simulink model "HvCoorn"  (R2022b)
settings: configuration reference "Icar05FusaMdlCfg" (kept outside this file)
undefined symbols (not defined in the file): BMSActSt_ACChrg, BMSActSt_DCChrg, BMSActSt_disconnect, BMSActSt_offline, BMSActSt_online, BMSActSt_undefined, BMSMainNegRlySt_Clsd_SC, BMSMainNegRlySt_Open_SC, BMSMainNegRlySt_StuckInClsd_SC, BMSMainNegRlySt_StuckInOpen_SC, BMSMainPosRlySt_Clsd_SC, BMSMainPosRlySt_Open_SC, BMSMainPosRlySt_StuckInClsd_SC, BMSPrecRlySt_StuckInOpen_SC, BMSReqSt_ACChrg, BMSReqSt_DCChrg, BMSReqSt_emergencyOffline, BMSReqSt_offline, BMSReqSt_online, Chrg_stCycleBookMod_SC, Chrg_stSingleBookMod_SC, CmpgMod_stInactv_SC, DCDCActSt_buck, DCDCActSt_connected, DCDCActSt_disconnected, DCDCReqSt_buck, DCDCReqSt_standby, EngStrtStop_RefuModDft_SC, EPBActSt_Appld_SC, GearLvr_stDrvGearD_SC, GearLvr_stDrvGearN_SC, GearLvr_stDrvGearP_SC, GearLvr_stDrvGearR_SC, hpp_bACChargeLinkIni_C, hpp_bACChargeLinkOKIni_C, hpp_bAcChgEnaIni_C, hpp_bAcChgPauseIni_C, hpp_bAcLinkTempErrIni_C, hpp_bBattWarmReqIni_C, hpp_bHvilHwErrIni_C, hpp_bHvilStOkIni_C, hpp_bHvRelayClsActIni_C, hpp_bHvRelayOpnActIni_C, hpp_bHvRelayStuckIni_C, hpp_bParked4ChDchgIni_C, hpp_bRemLvBatMntnReqIni_C, hpp_bStartUpReqIni_C, hpp_stHvilCanIni_C, hpp_stWarmTimeCfgRespIni_C, HvCoorn_bAuthEnaSwt_C, HvCoorn_bAuthFailSpdLimOvrd_C, HvCoorn_bAuthFailSpdLimOvrdVal_C, HvCoorn_bAuthStrt_C, HvCoorn_bBMSUnexpdDcnctFailEna_C, HvCoorn_bBuck2RdyBypDCDCEna_C, HvCoorn_bDCChrgFctCfg_C, HvCoorn_bDcChrgWkupEnaChrgLink_C, HvCoorn_bDCDcnct4ACEna_C, HvCoorn_bDCNotBuck2ShtdwnEna_C, HvCoorn_bDrvrLevNotRdyEna_C ... (+295)
libraries: ITKLib x213, simulink x61
(part 3 of 12)

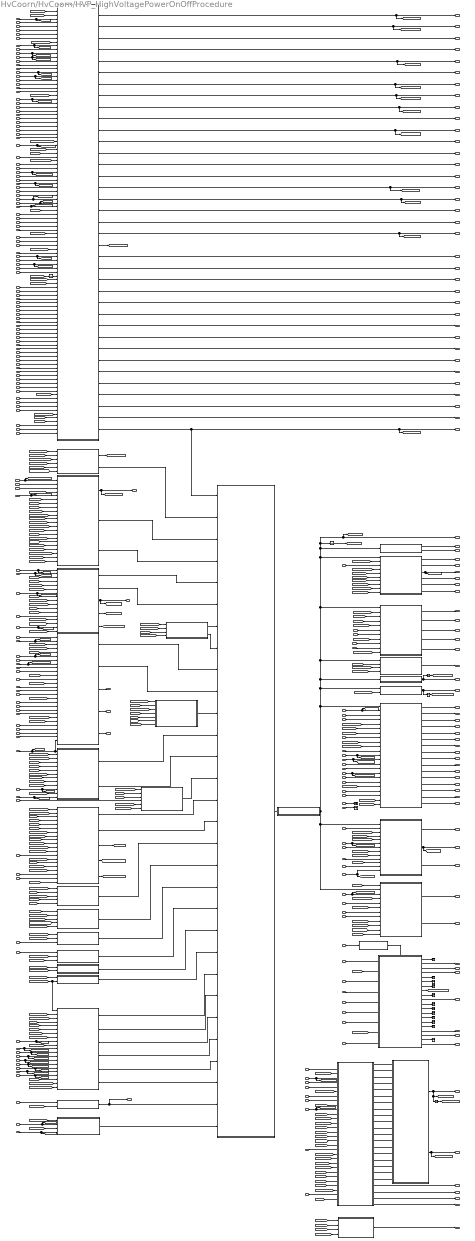
== system HvCoorn/HvCoorn/HVP_HighVoltagePowerOnOffProcedure ==
  idi_bKeyOn : Inport
  ian_uSupBattVolt : Inport  Port=2
  ian_tAcChrgrL1Temp : Inport  Port=3
  ian_tAcChrgrNTemp : Inport  Port=4
  ian_tDcChrgrTemp1 : Inport  Port=5
  ian_tDcChrgrTemp2 : Inport  Port=6
  icbms_bDcChrgWkup : Inport  Port=7
  icbms_bPrecResOverTemp : Inport  Port=8
  icbms_iHVBat : Inport  Port=9
  icbms_uHVBat : Inport  Port=10
  icbms_bBatACChrgFull : Inport  Port=11  OutDataTypeStr=boolean
  icbms_bStHvilSigErr : Inport  Port=12  OutDataTypeStr=boolean
  icbms_stHvBat : Inport  Port=13
  icbms_stHvil : Inport  Port=14  OutDataTypeStr=uint8
  icbms_stMainNegRly : Inport  Port=15  OutDataTypeStr=uint8
  icbms_stMainPosRly : Inport  Port=16  OutDataTypeStr=uint8
  icbms_stPrecRly : Inport  Port=17  OutDataTypeStr=uint8
  icbms_stDcChrgrCnct : Inport  Port=18
  icbms_bBatDCChrgFull : Inport  Port=19
  icbms_uDcChgrCap : Inport  Port=20
  icbms_iDcChgrCap : Inport  Port=21
  icecc_bStalHeatReq : Inport  Port=22
  icrm_stPlsHeatg : Inport  Port=23
  icrm_stStalHeatg : Inport  Port=24
  icbms_stDcChrg : Inport  Port=25
  icbms_bDcChrgCfg : Inport  Port=26
  icdc_bUHvActSigErr : Inport  Port=27
  icdc_stMode : Inport  Port=28
  icdc_uHvAct : Inport  Port=29
  icdc_bStHvilSigErr : Inport  Port=30  OutDataTypeStr=boolean
  icdc_stHvil : Inport  Port=31  OutDataTypeStr=uint8
  icfm_bUActSigErr : Inport  Port=32
  icfm_nAct : Inport  Port=33
  icfm_stMode : Inport  Port=34
  icfm_stActvDchrg : Inport  Port=35
  icfm_uAct : Inport  Port=36
  icrm_bUActSigErr : Inport  Port=37
  icrm_nAct : Inport  Port=38
  icrm_stMode : Inport  Port=39
  icrm_stActvDchrg : Inport  Port=40
  icrm_uAct : Inport  Port=41
  icobc_bUHvDcActSigErr : Inport  Port=42
  icobc_stChrgrCnct : Inport  Port=43
  icobc_stOBCMode : Inport  Port=44
  icobc_uHvDcAct : Inport  Port=45
  icobc_bChrgrCtrlSigCnct : Inport  Port=46  OutDataTypeStr=boolean
  icobc_bStAcHvilSigErr : Inport  Port=47  OutDataTypeStr=boolean
  icobc_pwrChrgMax : Inport  Port=48
  icobc_stHvil : Inport  Port=49  OutDataTypeStr=uint8
  icobc_uChrgrCtrlSigVolt : Inport  Port=50
  idi_bKeyStrt : Inport  Port=51
  BrkPedDev_bBrk : Inport  Port=52
  idi_bHvilInput : Inport  Port=53  OutDataTypeStr=boolean
  icacu_stWarmTime : Inport  Port=54  OutDataTypeStr=uint8
  icepb_stEpbSys : Inport  Port=55  OutDataTypeStr=uint8
  iczcu_stRmtChrgReq : Inport  Port=56
  Chrg_stBookChrgMod : Inport  Port=57  OutDataTypeStr=uint8
  ictel_stHvBatPrecdng : Inport  Port=58  OutDataTypeStr=uint8
  inv_stHvBattWarmTime : Inport  Port=59
  iud_stVCUImmo : Inport  Port=60
  iud_bNoHVHWarmTiCfg : Inport  Port=61  OutDataTypeStr=boolean
  iud_bNoHVHConfig : Inport  Port=62  OutDataTypeStr=boolean
  iud_stOBCWakeUpOrigin : Inport  Port=63  OutDataTypeStr=uint8
  iud_stRemoteImmo : Inport  Port=64  OutDataTypeStr=uint8
  PwrLimBatt_pwrMaxHvesDChrg : Inport  Port=65
  GearLvr_stDrvGear : Inport  Port=66
  VehSpd_vVeh : Inport  Port=67
  Chrg_stChrg : Inport  Port=68
  Chrg_bACChrgCmpl : Inport  Port=69  OutDataTypeStr=boolean
  Chrg_bDCChrgCmpl : Inport  Port=70
  std_tExterTemp : Inport  Port=71
  tcj_bHvBatPrecdngFinish : Inport  Port=72  OutDataTypeStr=boolean
  VehCfg_bFrntMotByp : Inport  Port=73
  Chrg_bChrgErrForever : Inport  Port=74
  icbms_bHvShutOffReq : Inport  Port=75
  iczcu_bHVPwrOffReq : Inport  Port=76
  icbms_bPlsHeatReq : Inport  Port=77
  icecc_bHVReq : Inport  Port=78
  icbms_uDCLnk : Inport  Port=79
  icbms_stPrechrgMod : Inport  Port=80
  DTC_bDiagRst : Inport  Port=81
  DTC_bDiagEnaCdnWkupLong : Inport  Port=82
  ipf_bPCAN0x130Vld : Inport  Port=83
  ipf_bPCAN0x111S1Vld : Inport  Port=84
  ipf_bPCAN0x110S1Vld : Inport  Port=85
  ipf_bPCANBusOffErr : Inport  Port=86
  icecc_bWPTCHvilFlt : Inport  Port=87
  icecc_bEASHvilFlt : Inport  Port=88
  ipf_bPCAN0x353Vld : Inport  Port=89
  DTC_bDiagEnaCdnWkupSho : Inport  Port=90
  iczcu_stFMCUAuthent : Inport  Port=91
  DrvMod_bVehShowMod : Inport  Port=92
  icicm_bPwrOffReq : Inport  Port=93
  icisg_nAct : Inport  Port=94
  ved_bInhbHvOn : Inport  Port=95
  ved_bInhbRdy : Inport  Port=96
  ved_bHvShtdwn : Inport  Port=97
  ved_bEmgcyHvShtdwn : Inport  Port=98
  ipf_bBD1CAN0x41CVld : Inport  Port=99
  icbms_stIsolTst : Inport  Port=100
  icicm_bOTAOn : Inport  Port=101
  icicm_stHVReq : Inport  Port=102
  icobc_bDchrgrCnct : Inport  Port=103
  ictcp_stRmtHvReq : Inport  Port=104
  icicm_stIvtrSwt : Inport  Port=105
  icbms_pctHVBatSOCDisp : Inport  Port=106
  icicm_pctSOCV2XLimSet : Inport  Port=107
  HvGrid_pwrMotDChrgMax : Inport  Port=108
  iczcu_stCarMod : Inport  Port=109
  ParkCtrl_bRPAActv : Inport  Port=110
  icbms_stChrgSts : Inport  Port=111
  ipf_bPCAN0x343S2Vld : Inport  Port=112
  HvCoorn_pctSOCV2XLimSetEER : Inport  Port=113
  Chrg_bChrgStopBySOCLim : Inport  Port=114
  Chrg_bBookChrgCmpl : Inport  Port=115
  iud_bNetMaintn : Inport  Port=116
  icobc_bVehCnct : Inport  Port=117
  icisg_uAct : Inport  Port=118
  icisg_stMod : Inport  Port=119
  icdkm_stLrcpReq : Inport  Port=120
  ictcp_stLostComWarn : Inport  Port=121
  iczcu_stRMCUAuthent : Inport  Port=122
  icfm_bHvilFlt : Inport  Port=123
  icrm_bHvilFlt : Inport  Port=124
  PwrLimBatt_pwrContnsDChrg : Inport  Port=125
  icicm_stIvtrEnaSwt : Inport  Port=126
  ibsw_bCnctElecDvce : Inport  Port=127
  ipf_bPCAN0x340S1Vld : Inport  Port=128
  icbms_bIsolFlt : Inport  Port=129
  DTC_bBMSFltLvlOver5 : Inport  Port=130
  icems_stEng : Inport  Port=131
  GearLvr_bNapModActv : Inport  Port=132
  GearLvr_stCmpgMod : Inport  Port=133
  GearLvr_bOffVehPwrKeep : Inport  Port=134
  GearLvr_bSentilMod : Inport  Port=135
  icebs_pctLvBatSoh : Inport  Port=136
  icbms_tMaxBat : Inport  Port=137
  icbms_tMinBat : Inport  Port=138
  icebs_tLvBat : Inport  Port=139
  icebs_pctLvBatSoc : Inport  Port=140
  icebs_stSocPrcsn : Inport  Port=141
  icebs_uLvBat : Inport  Port=142
  icicm_stOTAPwrMngtReq : Inport  Port=143
  HvCoorn_ctSmtBatMntnFailEER : Inport  Port=144
  iud_bEEIniFnsd : Inport  Port=145
  HvCoorn_ctSmtBatMntnSucsEER : Inport  Port=146
  iclbms_stLvRemChrgReq : Inport  Port=147
  ipf_bLBMSCANVld : Inport  Port=148
  VehCfg_stLvBattTyp : Inport  Port=149
  icems_nAct : Inport  Port=150
  EngStrtStop_bFuChrgActvEEW : Inport  Port=151
  icobc_stOBCModeV2In : Inport  Port=152
  icisg_bHvilFlt : Inport  Port=153
  VCU_E2_counterfaieldEER : Inport  Port=154
  VCCM_flg_Allow_Antitheft : Inport  Port=155
  VCCM_flg_Antitheft_Overtime : Inport  Port=156
  VCCM_flg_Antitheft_Start : Inport  Port=157
  ictcp_noAuthChlgOnReq : Inport  Port=158
  ictcp_noAuthSts : Inport  Port=159
  VCCM_flg_SK_Recep_ok : Inport  Port=160
  idi_uPwrSply : Inport  Port=161
  EngStrtStop_bHVPRdy : Inport  Port=162
  DTC_bBMSFltLvl6 : Inport  Port=163
  DTC_bBMSFltLvl7 : Inport  Port=164
  DTC_bBMSFltLvl8 : Inport  Port=165
  EngStrtStop_bEngStrtAllw : Inport  Port=166
  HybCoorn_bEngStrtFail : Inport  Port=167
  ved_bInhbEngStrt : Inport  Port=168
  ipf_bLIN9EBS0x34NodLostErr : Inport  Port=169
  DTC_bBMSFltLvl5 : Inport  Port=170
  EngStrtStop_stRefuMod : Inport  Port=171
  VehCfg_stCycCdn : Inport  Port=172
  icbcm_stDrvrSeatBelt : Inport  Port=173
  icbcm_bStDrvrSeatBeltSigErr : Inport  Port=174
  icbcm_bDrvrDoorAjar : Inport  Port=175
  icbcm_bDrvrDoorAjarSigErr : Inport  Port=176
  HvGrid_pwrLoadAct : Inport  Port=177
  HvCoorn_bSocWkupEER : Inport  Port=178
  HvCoorn_bTimerWkupReqEER : Inport  Port=179
  icobc_stV2LFltTyp : Inport  Port=180
  HvCoorn_stRemLvBatMntnFailRsnEER : Inport  Port=181
  icems_bFanAftRunActv : Inport  Port=182
  RngPrdn_volFuRmnByInstModEEW : Inport  Port=183
  idi_bEBSLinWkup : Inport  Port=184
  idi_bTimerWkup : Inport  Port=185
  HvCoorn_pctHVBatSocEER : Inport  Port=186
  idi_noBMSSocCounter : Inport  Port=187
  icecc_uPTCAct : Inport  Port=188
  icecc_uEASAct : Inport  Port=189
  ved_bCellVoltUndLimSrus : Inport  Port=190
  A01_HighvoltPowerUpReq : Subsystem
  A02_Init2StupCal : Subsystem  Description=初始化跳转至上高压
  A03_Comm2HVReqCal : Subsystem  Description=通讯连接跳转至高压请求
  A04_HVReq2DCBuckCal : Subsystem  Description=高压请求跳转至DCDC Buck
  A05_DCDCBuck2ReadyCal : Subsystem  Description=DCDC Buck跳转至高压Ready
  A06_ReadyWait2ReadyCal : Subsystem  Description=Ready Wait跳转至Ready
  A07_MindChange2ReadyCal : Subsystem  Description=MindChange跳转至Ready
  A08_MindChange2ShutHVCal : Subsystem  Description=MindChange跳转至断高压
  A09_ShutHV2ShutDisChCal : Subsystem  Description=断高压跳转至主动放电
  A10_ShutDisCh2ShutECUCal : Subsystem  Description=主动放电跳转至关ECU
  A11_ShutECU2AftRunCal : Subsystem  Description=关断ECU跳转至后运行
  A12_ShutECU2CommCal : Subsystem  Description=关断ECU跳转至通讯准备
  A13_AftRun2NetManCal : Subsystem  Description=后运行跳转至网络保持
  A14_NetMan2PwrShutCal : Subsystem  Description=后运行跳转至网络保持
  A15_Wake2NetManCal : Subsystem  Description=唤醒跳转至网络保持
  A16_Init2AftRunCal : Subsystem  Description=初始化跳转至后运行
  A17_EmergencyShutDownCal : Subsystem  Description=紧急下电
  A18_ShutDownReqCal : Subsystem  Description=故障下高压
  A19_MainProcedure : Stateflow chart  TreatAsAtomicUnit=on
      settings: PortSchema="{\"entries\":[{\"content\":{\"sides\":[{\"content\":{\"connectorIds\":[\"In1\",\"In2\",\"In3\",\"In4\",\"In5\",\"In6\",\"In7\",\"In8\",\"In9\",\"In10\",\"In11\",\"In12\",\"In29\",\"In13\",\"In14\",\"In15\",\"In16\",\"In17\",\"In18\",\"In19\",\"In20\",\"In21\",\"In22\",\"In23\",\"In24\",\"In25\",\"In26\",\"In27\",\"In28\",\"In30\"]},\"type\":\"ConnectorPlacement.EquallySpacedRectSide\",\"uuid\":\"b4d08740-7c56-442d-9e50-6eb0ed517615\"},{\"content\":{\"connectorIds\":[\"Out1\"],\"side\":\"RIGHT\"},\"type\":\"ConnectorPlacement.EquallySpacedRectSide\",\"uuid\":\"58ee4b8b-9875-4a72-814f-6ccb341ac7ee\"},{\"content\":{\"connectorIds\":[],\"side\":\"TOP\"},\"type\":\"ConnectorPlacement.EquallySpacedRectSide\",\"uuid\":\"584c371a-54d2-4cc4-a7a6-7136bc7e8093\"}]},\"type\":\"ConnectorPlacement.EquallySpacedConnector\",\"uuid\":\"c86f169c-7c4a-42d5-917a-7ec3533626c8\"}],\"packageUris\":[\"http://schema.mathworks.com/mf0/Connector/R2020b\"],\"version\":\"1.0\"}"
  A20_HVPStOvrd : Subsystem
  A21_ShutDwnEna : Subsystem
  A22_ModeBMSReqCal : Subsystem  Description=电池模式请求
  A23_MCUModeReqCal : Subsystem  Description=电机模式请求
  A24_DCDCModeReqCal : Subsystem  Description=DCDC模式请求
  A25_HvilClsReqCal : Subsystem
  A26_DischargeErrCal : Subsystem  Description=主动放电故障
  A27_ErrCheck : Subsystem
  A28_V2L : Subsystem
  A29_V2In : Subsystem
  A30_Authcation : Subsystem
  A30_ISGNotRdy : Subsystem
  A31_VoltModReq : Subsystem
  A32_VoltModSts : Stateflow chart  TreatAsAtomicUnit=on
  A33_ISGVoltReq : Subsystem
  Subsystem : Subsystem
  Terminator{,1..13} (14 alike) : Terminator
  Unit Delay{1..4} (4 alike) : UnitDelay  SampleTime=-1  HasFrameUpgradeWarning=on
      Unit Delay1 settings: AttributesFormatString=<initial=%<X0>>
      Unit Delay2 settings: AttributesFormatString=<initial=%<X0>>
      Unit Delay3 settings: AttributesFormatString=<initial=%<X0>>
      Unit Delay4 settings: AttributesFormatString=<initial=%<x0>>
  UnitDelay : UnitDelay  SampleTime=-1  HasFrameUpgradeWarning=on
      settings: AttributesFormatString=<Initial=%<x0>>
  HvCoorn_stHVP : Outport  VectorParamsAs1DForOutWhenUnconnected=off
  HvCoorn_stFMCUModeReq : Outport  Port=2  VectorParamsAs1DForOutWhenUnconnected=off
  HvCoorn_stRMCUModeReq : Outport  Port=3  VectorParamsAs1DForOutWhenUnconnected=off
  HvCoorn_stDCDCModeReq : Outport  Port=4  VectorParamsAs1DForOutWhenUnconnected=off
  HvCoorn_bHvOnReq : Outport  Port=5  VectorParamsAs1DForOutWhenUnconnected=off
  HvCoorn_stBMSModeReq : Outport  Port=6  VectorParamsAs1DForOutWhenUnconnected=off
  HvCoorn_bHvilClsReq : Outport  Port=7  VectorParamsAs1DForOutWhenUnconnected=off
  HvCoorn_bActvDischargeErr : Outport  Port=8  VectorParamsAs1DForOutWhenUnconnected=off
  HvCoorn_bEmgcyShutDownReq : Outport  Port=9  VectorParamsAs1DForOutWhenUnconnected=off
  HvCoorn_bHvOnFail : Outport  Port=10  VectorParamsAs1DForOutWhenUnconnected=off
  HvCoorn_bHvInitFail : Outport  Port=11  VectorParamsAs1DForOutWhenUnconnected=off
  HvCoorn_bHvReady : Outport  Port=12  VectorParamsAs1DForOutWhenUnconnected=off
  HvCoorn_bDrvRdy : Outport  Port=13  VectorParamsAs1DForOutWhenUnconnected=off
  HvCoorn_bACChrgLink : Outport  Port=14  InitialOutput=hpp_bACChargeLinkIni_C  VectorParamsAs1DForOutWhenUnconnected=off
  HvCoorn_bACChrgLinkOk : Outport  Port=15  InitialOutput=hpp_bACChargeLinkOKIni_C  VectorParamsAs1DForOutWhenUnconnected=off
  HvCoorn_stHvil : Outport  Port=16  InitialOutput=hpp_stHvilCanIni_C  VectorParamsAs1DForOutWhenUnconnected=off
  HvCoorn_bHvilHwErr : Outport  Port=17  InitialOutput=hpp_bHvilHwErrIni_C  VectorParamsAs1DForOutWhenUnconnected=off
  HvCoorn_bHvilStOk : Outport  Port=18  InitialOutput=hpp_bHvilStOkIni_C  VectorParamsAs1DForOutWhenUnconnected=off
  HvCoorn_bACChrgPause : Outport  Port=19  InitialOutput=hpp_bAcChgPauseIni_C  VectorParamsAs1DForOutWhenUnconnected=off
  HvCoorn_bStartUpReq : Outport  Port=20  InitialOutput=hpp_bStartUpReqIni_C  VectorParamsAs1DForOutWhenUnconnected=off
  HvCoorn_bHvRlyClsAct : Outport  Port=21  InitialOutput=hpp_bHvRelayClsActIni_C  VectorParamsAs1DForOutWhenUnconnected=off
  HvCoorn_bHvRlyOpenAct : Outport  Port=22  InitialOutput=hpp_bHvRelayOpnActIni_C  VectorParamsAs1DForOutWhenUnconnected=off
  HvCoorn_bHvRlyStuck : Outport  Port=23  InitialOutput=hpp_bHvRelayStuckIni_C  VectorParamsAs1DForOutWhenUnconnected=off
  HvCoorn_bACLinkTempErr : Outport  Port=24  InitialOutput=hpp_bAcLinkTempErrIni_C  VectorParamsAs1DForOutWhenUnconnected=off
  HvCoorn_bParked4ChDchg : Outport  Port=25  InitialOutput=hpp_bParked4ChDchgIni_C  VectorParamsAs1DForOutWhenUnconnected=off
  HvCoorn_bBattWarmReq : Outport  Port=26  InitialOutput=hpp_bBattWarmReqIni_C  VectorParamsAs1DForOutWhenUnconnected=off
  HvCoorn_stWarmTimeCfgResp : Outport  Port=27  InitialOutput=hpp_stWarmTimeCfgRespIni_C  VectorParamsAs1DForOutWhenUnconnected=off
  HvCoorn_bACChrgEna : Outport  Port=28  InitialOutput=hpp_bAcChgEnaIni_C  VectorParamsAs1DForOutWhenUnconnected=off
  HvCoorn_bRemLvBatMntnReq : Outport  Port=29  InitialOutput=hpp_bRemLvBatMntnReqIni_C  VectorParamsAs1DForOutWhenUnconnected=off
  HvCoorn_bDCChrgLink : Outport  Port=30  VectorParamsAs1DForOutWhenUnconnected=off
  HvCoorn_bChrgLink : Outport  Port=31  VectorParamsAs1DForOutWhenUnconnected=off
  HvCoorn_bDCLinkTempErr : Outport  Port=32  VectorParamsAs1DForOutWhenUnconnected=off
  HvCoorn_bDCChrgEna : Outport  Port=33  VectorParamsAs1DForOutWhenUnconnected=off
  HvCoorn_bRMCUPlsHeatgReq : Outport  Port=34
  HvCoorn_bRMCUStalHeatgReq : Outport  Port=35
  HvCoorn_bEccEna : Outport  Port=36  VectorParamsAs1DForOutWhenUnconnected=off
  HvCoorn_bHvRlyUnexpdDcnctErr : Outport  Port=37
  HvCoorn_bBMSUnexpdDcnctErr : Outport  Port=38
  HvCoorn_bMainRlyFail2ClsErr : Outport  Port=39
  HvCoorn_bPrechrgOvtiErr : Outport  Port=40
  HvCoorn_bDchrgOvtiErr : Outport  Port=41
  HvCoorn_bDCUnexpdDcnctErr : Outport  Port=42
  HvCoorn_stISGModeReq : Outport  Port=43  VectorParamsAs1DForOutWhenUnconnected=off
  HvCoorn_stStartUpReq : Outport  Port=44  VectorParamsAs1DForOutWhenUnconnected=off
  HvCoorn_bV2LReq : Outport  Port=45  VectorParamsAs1DForOutWhenUnconnected=off
  HvCoorn_bV2LActv : Outport  Port=46  VectorParamsAs1DForOutWhenUnconnected=off
  HvCoorn_bAllwShutNet : Outport  Port=47
  HvCoorn_bAllwSlep : Outport  Port=48
  HvCoorn_pctSOCV2XLimSetEEW : Outport  Port=49  VectorParamsAs1DForOutWhenUnconnected=off
  HvCoorn_stRdy2RdyWait : Outport  Port=50  VectorParamsAs1DForOutWhenUnconnected=off
  HvCoorn_bAuthentPass : Outport  Port=51  VectorParamsAs1DForOutWhenUnconnected=off
  HvCoorn_bBMSHvilErr : Outport  Port=52  VectorParamsAs1DForOutWhenUnconnected=off
  HvCoorn_bFMCUHvilErr : Outport  Port=53  VectorParamsAs1DForOutWhenUnconnected=off
  HvCoorn_bRMCUHvilErr : Outport  Port=54  VectorParamsAs1DForOutWhenUnconnected=off
  HvCoorn_bOBCHvilErr : Outport  Port=55  VectorParamsAs1DForOutWhenUnconnected=off
  HvCoorn_bDCDCHvilErr : Outport  Port=56  VectorParamsAs1DForOutWhenUnconnected=off
  HvCoorn_bHWHvilErr : Outport  Port=57  VectorParamsAs1DForOutWhenUnconnected=off
  HvCoorn_bWPTCHvilErr : Outport  Port=58  VectorParamsAs1DForOutWhenUnconnected=off
  HvCoorn_bEASHvilErr : Outport  Port=59  VectorParamsAs1DForOutWhenUnconnected=off
  HvCoorn_bMCUAuthentPass : Outport  Port=60  VectorParamsAs1DForOutWhenUnconnected=off
  HvCoorn_bV2InReq : Outport  Port=61  VectorParamsAs1DForOutWhenUnconnected=off
  HvCoorn_bV2InEna : Outport  Port=62  VectorParamsAs1DForOutWhenUnconnected=off
  HvCoorn_bBMSIsoErr : Outport  Port=63  VectorParamsAs1DForOutWhenUnconnected=off
  HvCoorn_bKeyOnPwrUp : Outport  Port=64  VectorParamsAs1DForOutWhenUnconnected=off
  HvCoorn_bSocWkup : Outport  Port=65  VectorParamsAs1DForOutWhenUnconnected=off
  HvCoorn_ctSmtBatMntnFailEEW : Outport  Port=66  VectorParamsAs1DForOutWhenUnconnected=off
  HvCoorn_stRemLvBatMntnFailRsn : Outport  Port=67  VectorParamsAs1DForOutWhenUnconnected=off
  HvCoorn_ctSmtBatMntnSucsEEW : Outport  Port=68  VectorParamsAs1DForOutWhenUnconnected=off
  HvCoorn_bTimerWkupReq : Outport  Port=69  VectorParamsAs1DForOutWhenUnconnected=off
  HvCoorn_bLbmsLvBatMntnReq : Outport  Port=70  VectorParamsAs1DForOutWhenUnconnected=off
  HvCoorn_pctLbmsSocMntnThd : Outport  Port=71  VectorParamsAs1DForOutWhenUnconnected=off
  HvCoorn_bLbmsSocWkup : Outport  Port=72  VectorParamsAs1DForOutWhenUnconnected=off
  HvCoorn_bISGHvilErr : Outport  Port=73  VectorParamsAs1DForOutWhenUnconnected=off
  HvCoorn_bAntiTrig430 : Outport  Port=74  VectorParamsAs1DForOutWhenUnconnected=off
  HvCoorn_bAntiTrig42C : Outport  Port=75  VectorParamsAs1DForOutWhenUnconnected=off
  VCU_E2_counterfaieldEEW : Outport  Port=76  VectorParamsAs1DForOutWhenUnconnected=off
  HvCoorn_stAuthChkFailLvl : Outport  Port=77  VectorParamsAs1DForOutWhenUnconnected=off
  HvCoorn_noVcuAuthFb : Outport  Port=78  VectorParamsAs1DForOutWhenUnconnected=off
  HvCoorn_noVcuAuthReq : Outport  Port=79  VectorParamsAs1DForOutWhenUnconnected=off
  HvCoorn_bAuthFailSpdLim : Outport  Port=80  VectorParamsAs1DForOutWhenUnconnected=off
  HvCoorn_bVehNetWkupEna : Outport  Port=81  VectorParamsAs1DForOutWhenUnconnected=off
  HvCoorn_stVoltMod : Outport  Port=82  VectorParamsAs1DForOutWhenUnconnected=off
  HvCoorn_bVoltModStbReq : Outport  Port=83  VectorParamsAs1DForOutWhenUnconnected=off
  HvCoorn_bVoltModHvDisbOvtiErr : Outport  Port=84  VectorParamsAs1DForOutWhenUnconnected=off
  HvCoorn_bVoltModHvDcnctOvtiErr : Outport  Port=85  VectorParamsAs1DForOutWhenUnconnected=off
  HvCoorn_bVoltModHvReqOvtiErr : Outport  Port=86  VectorParamsAs1DForOutWhenUnconnected=off
  HvCoorn_uISGReq : Outport  Port=87  VectorParamsAs1DForOutWhenUnconnected=off
  HvCoorn_bRdyLamp : Outport  Port=88
  HvCoorn_bSocWkupEEW : Outport  Port=89  VectorParamsAs1DForOutWhenUnconnected=off
  HvCoorn_bTimerWkupReqEEW : Outport  Port=90  VectorParamsAs1DForOutWhenUnconnected=off
  HvCoorn_stRemLvBatMntnFailRsnEEW : Outport  Port=91  VectorParamsAs1DForOutWhenUnconnected=off
  HvCoorn_pctHVBatSocEEW : Outport  Port=92  VectorParamsAs1DForOutWhenUnconnected=off
  HvCoorn_bDft2EngStrtRaw : Outport  Port=93  VectorParamsAs1DForOutWhenUnconnected=off
  HvCoorn_bShowModSocLo : Outport  Port=94  VectorParamsAs1DForOutWhenUnconnected=off
  wires:
  Unit Delay2/1 -> [HvCoorn_stHVPOld]  "HvCoorn_stHVPOld"
  [HvCoorn_stHVPOld] -> A02_Init2StupCal/5(HvCoorn_stHVPOld)
  A02_Init2StupCal/2(HvCoorn_bInit2StrtUp) -> A19_MainProcedure/2(HvCoorn_bInit2StrtUp)
  A05_DCDCBuck2ReadyCal/1(HvCoorn_bDCBuck2Rdy) -> A19_MainProcedure/7(HvCoorn_bDCBuck2Rdy)
  A07_MindChange2ReadyCal/1(HvCoorn_bMindChag2Rdy) -> A19_MainProcedure/11(HvCoorn_bMindChag2Rdy)
  A08_MindChange2ShutHVCal/1(HvCoorn_bMindChag2ShutHV) -> A19_MainProcedure/12(HvCoorn_bMindChag2ShutHV)
  A11_ShutECU2AftRunCal/1(HvCoorn_bShutECU2AftRun) -> A19_MainProcedure/16(HvCoorn_bShutECU2AftRun)
  A13_AftRun2NetManCal/1(HvCoorn_bAftRun2NetMan) -> A19_MainProcedure/18(HvCoorn_bAftRun2NetMan)
  A16_Init2AftRunCal/1(HvCoorn_bInit2AftRun) -> A19_MainProcedure/21(HvCoorn_bInit2AftRun)
  A18_ShutDownReqCal/1(HvCoorn_bEmgcyShutDownReq) -> HvCoorn_bEmgcyShutDownReq/1, A19_MainProcedure/28(HvCoorn_bEmgcyShutDownReq)
  icdc_stMode/1 -> A01_HighvoltPowerUpReq/17(icdc_stMode), [icdc_stMode]
  icfm_uAct/1 -> A04_HVReq2DCBuckCal/1(icfm_uAct), [icfm_uAct]
  [HvCoorn_bStartUpReq] -> A05_DCDCBuck2ReadyCal/2(HvCoorn_bStartUpReq)
  [HvCoorn_bStartUpReq] -> A07_MindChange2ReadyCal/1(HvCoorn_bStartUpReq)
  icbms_iHVBat/1 -> A08_MindChange2ShutHVCal/11(icbms_iHVBat), [icbms_iHVBat]
  [icfm_stMode] -> A07_MindChange2ReadyCal/2(icfm_stMode)
  [icfm_stMode] -> A08_MindChange2ShutHVCal/4(icfm_stMode)
  [icdc_stMode] -> A08_MindChange2ShutHVCal/6(icdc_stMode)
  [HvCoorn_bStartUpReq] -> A15_Wake2NetManCal/1(HvCoorn_bStartUpReq)
  [HvCoorn_bStartUpReq] -> A16_Init2AftRunCal/1(HvCoorn_bStartUpReq)
  [icfm_uAct] -> A11_ShutECU2AftRunCal/2(icfm_uAct)
  [HvCoorn_bHvRlyOpenAct] -> A17_EmergencyShutDownCal/3(HvCoorn_bHvRlyOpenAct)
  [icfm_uAct] -> A17_EmergencyShutDownCal/4(icfm_uAct)
  A25_HvilClsReqCal/1(HvCoorn_bHvilClsReq) -> Unit Delay3/1, HvCoorn_bHvilClsReq/1
  A12_ShutECU2CommCal/1(HvCoorn_bShutECU2Comm) -> A19_MainProcedure/17(HvCoorn_bShutECU2Comm)
  [HvCoorn_bStartUpReq] -> A13_AftRun2NetManCal/2(HvCoorn_bStartUpReq)
  [HvCoorn_bStartUpReq] -> A02_Init2StupCal/1(HvCoorn_bStartUpReq)
  icfm_stMode/1 -> A01_HighvoltPowerUpReq/18(icfm_stMode), [icfm_stMode]
  [icdc_uHvAct] -> A17_EmergencyShutDownCal/5(icdc_uHvAct)
  [HvCoorn_bHvRlyOpenAct] -> A09_ShutHV2ShutDisChCal/1(HvCoorn_bHvRlyOpenAct)
  idi_bKeyStrt/1 -> [idi_bKeyStrt], A06_ReadyWait2ReadyCal/2(idi_bKeyStrt)
  A23_MCUModeReqCal/1(HvCoorn_stFMCUModeReq) -> HvCoorn_stFMCUModeReq/1
  A26_DischargeErrCal/1(HvCoorn_bActvDischargeErr) -> HvCoorn_bActvDischargeErr/1, Unit Delay1/1
  A24_DCDCModeReqCal/1(HvCoorn_stDCDCModeReq) -> HvCoorn_stDCDCModeReq/1
  A22_ModeBMSReqCal/1(HvCoorn_bHvOnReq) -> HvCoorn_bHvOnReq/1
  [HvCoorn_bStartUpReq] -> A26_DischargeErrCal/2(HvCoorn_bStartUpReq)
  ian_uSupBattVolt/1 -> A03_Comm2HVReqCal/2(ian_uSupBattVolt)
  [HvCoorn_bStartUpReq] -> A08_MindChange2ShutHVCal/7(HvCoorn_bStartUpReq)
  A03_Comm2HVReqCal/2(HvCoorn_bComm2HVReq) -> A19_MainProcedure/3(HvCoorn_bComm2HVReq)
  A04_HVReq2DCBuckCal/2(HvCoorn_bHVReq2ShutDown) -> A19_MainProcedure/6(HvCoorn_bHVReq2ShutDown)
  A04_HVReq2DCBuckCal/1(HvCoorn_bHVReq2DCBuck) -> A19_MainProcedure/5(HvCoorn_bHVReq2DCBuck)
  A04_HVReq2DCBuckCal/3(HvCoorn_bHvOnFail) -> HvCoorn_bHvOnFail/1, [HvCoorn_bHvOnFail]
  A06_ReadyWait2ReadyCal/2(HvCoorn_bRdy2RdyWait) -> A19_MainProcedure/10(HvCoorn_bRdy2RdyWait)
  A06_ReadyWait2ReadyCal/1(HvCoorn_bRdyWait2Rdy) -> A19_MainProcedure/9(HvCoorn_bRdyWait2Rdy)
  A10_ShutDisCh2ShutECUCal/2(HvCoorn_bShutDisCh2ShutErr) -> A19_MainProcedure/15(HvCoorn_bShutDisCh2ShutErr)
  A10_ShutDisCh2ShutECUCal/1(HvCoorn_bShutDisCh2ShutECU) -> A19_MainProcedure/14(HvCoorn_bShutDisCh2ShutECU)
  A14_NetMan2PwrShutCal/1(HvCoorn_bNetMan2PwrShut) -> A19_MainProcedure/19(HvCoorn_bNetMan2PwrShut)
  A15_Wake2NetManCal/1(HvCoorn_bWake2NetMan) -> A19_MainProcedure/20(HvCoorn_bWake2NetMan)
  A17_EmergencyShutDownCal/5(HvCoorn_bEmWaitKeyOff2NetMan) -> A19_MainProcedure/26(HvCoorn_bEmWaitKeyOff2NetMan)
  A17_EmergencyShutDownCal/4(HvCoorn_bEmDisCh2Err) -> A19_MainProcedure/25(HvCoorn_bEmDisCh2Err)
  A17_EmergencyShutDownCal/3(HvCoorn_bEmDisCh2WaitKeyOff) -> A19_MainProcedure/24(HvCoorn_bEmDisCh2WaitKeyOff)
  A17_EmergencyShutDownCal/2(HvCoorn_bEmShutHv2DisCh) -> A19_MainProcedure/23(HvCoorn_bEmShutHv2DisCh)
  A17_EmergencyShutDownCal/1(HvCoorn_bEmIni2ShutHV) -> A19_MainProcedure/22(HvCoorn_bEmIni2ShutHV)
  icbms_bPrecResOverTemp/1 -> A03_Comm2HVReqCal/3(icbms_bPrecResOverTemp)
  GearLvr_stDrvGear/1 -> A03_Comm2HVReqCal/5(GearLvr_stDrvGear), [GearLvr_stDrvGear]
  icobc_stOBCMode/1 -> A01_HighvoltPowerUpReq/24(icobc_stOBCMode), [icobc_stOBCMode]
  [HvCoorn_bHvilStOk] -> A03_Comm2HVReqCal/11(HvCoorn_bHvilStOk)
  [HvCoorn_bStartUpReq] -> A03_Comm2HVReqCal/12(HvCoorn_bStartUpReq)
  [HvCoorn_stHVPOld] -> A03_Comm2HVReqCal/14(HvCoorn_stHVPOld)
  [HvCoorn_bObcChrgrCnct] -> A03_Comm2HVReqCal/13(HvCoorn_bObcChrgrCnct)
  icdc_uHvAct/1 -> [icdc_uHvAct], A04_HVReq2DCBuckCal/2(icdc_uHvAct)
  [HvCoorn_stHVPOld] -> A04_HVReq2DCBuckCal/6(HvCoorn_stHVPOld)
  [HvCoorn_bStartUpReq] -> A04_HVReq2DCBuckCal/9(HvCoorn_bStartUpReq)
  [icfm_stMode] -> A04_HVReq2DCBuckCal/3(icfm_stMode)
  [icdc_stMode] -> A04_HVReq2DCBuckCal/4(icdc_stMode)
  [icobc_stOBCMode] -> A04_HVReq2DCBuckCal/5(icobc_stOBCMode)
  [idi_bKeyOn] -> A04_HVReq2DCBuckCal/8(idi_bKeyOn)
  [icdc_stMode] -> A05_DCDCBuck2ReadyCal/3(icdc_stMode)
  [icobc_stOBCMode] -> A08_MindChange2ShutHVCal/8(icobc_stOBCMode)
  [HvCoorn_bStartUpReq] -> A11_ShutECU2AftRunCal/3(HvCoorn_bStartUpReq)
  [HvCoorn_bHvOnFail] -> A02_Init2StupCal/2(HvCoorn_bHvOnFail)
  Unit Delay1/1 -> [HvCoorn_bDischargeErrOld]
  [HvCoorn_bDischargeErrOld] -> A02_Init2StupCal/3(HvCoorn_bDischargeErrOld)
  idi_bKeyOn/1 -> A01_HighvoltPowerUpReq/3(idi_bKeyOn), [idi_bKeyOn]
  A22_ModeBMSReqCal/2(HvCoorn_stBMSModeReq) -> HvCoorn_stBMSModeReq/1
  A03_Comm2HVReqCal/3(HvCoorn_bComm2ShutECU) -> A19_MainProcedure/4(HvCoorn_bComm2ShutECU)
  A03_Comm2HVReqCal/1(HvCoorn_bHvInitFail) -> [HvCoorn_bHvInitFail], HvCoorn_bHvInitFail/1
  [HvCoorn_bHvInitFail] -> A02_Init2StupCal/4(HvCoorn_bHvInitFail)
  [ved_bHvShtdwn] -> A08_MindChange2ShutHVCal/9(ved_bHvShtdwn)
  icfm_nAct/1 -> A17_EmergencyShutDownCal/9(icfm_nAct), [icfm_nAct]
  [icfm_stMode] -> A17_EmergencyShutDownCal/6(icfm_stMode)
  [icfm_nAct] -> A09_ShutHV2ShutDisChCal/2(icfm_nAct)
  [HvCoorn_bStartUpReq] -> A12_ShutECU2CommCal/2(HvCoorn_bStartUpReq)
  [HvCoorn_bHvOnFail] -> A12_ShutECU2CommCal/3(HvCoorn_bHvOnFail)
  [HvCoorn_bDischargeErrOld] -> A12_ShutECU2CommCal/4(HvCoorn_bDischargeErrOld)
  A10_ShutDisCh2ShutECUCal/3(bVolDiffEnaHv) -> [bVolDiffEnaHv]
  [HvCoorn_bHvInitFail] -> A12_ShutECU2CommCal/5(HvCoorn_bHvInitFail)
  [icdc_uHvAct] -> A11_ShutECU2AftRunCal/4(icdc_uHvAct)
  [icfm_uAct] -> A10_ShutDisCh2ShutECUCal/3(icfm_uAct)
  [icdc_uHvAct] -> A10_ShutDisCh2ShutECUCal/4(icdc_uHvAct)
  [icfm_stMode] -> A10_ShutDisCh2ShutECUCal/5(icfm_stMode)
  [HvCoorn_bStartUpReq] -> A10_ShutDisCh2ShutECUCal/7(HvCoorn_bStartUpReq)
  Chrg_stChrg/1 -> A22_ModeBMSReqCal/3(Chrg_stChrg)
  [Chrg_bACChrgCmpl] -> A22_ModeBMSReqCal/5(Chrg_bACChrgCmpl)
  [HvCoorn_bACChrgLinkOk] -> A22_ModeBMSReqCal/4(HvCoorn_bACChrgLinkOk)
  [icbms_iHVBat] -> A17_EmergencyShutDownCal/7(icbms_iHVBat)
  iud_stVCUImmo/1 -> A06_ReadyWait2ReadyCal/1(iud_stVCUImmo)
  [HvCoorn_bStartUpReq] -> A06_ReadyWait2ReadyCal/4(HvCoorn_bStartUpReq)
  [idi_bKeyOn] -> A06_ReadyWait2ReadyCal/5(idi_bKeyOn)
  [HvCoorn_stHVPOld] -> A18_ShutDownReqCal/2(HvCoorn_stHVPOld)
  A01_HighvoltPowerUpReq/37(HvCoorn_bStartUpReq) -> [HvCoorn_bStartUpReq], HvCoorn_bStartUpReq/1, A19_MainProcedure/1(HvCoorn_bStartUpReq)
  [HvCoorn_bHvRlyClsAct] -> A04_HVReq2DCBuckCal/10(HvCoorn_bHvRlyClsAct)
  [HvCoorn_bHvRlyClsAct] -> A07_MindChange2ReadyCal/3(HvCoorn_bHvRlyClsAct)
  VehSpd_vVeh/1 -> A06_ReadyWait2ReadyCal/28(VehSpd_vVeh), A08_MindChange2ShutHVCal/1(VehSpd_vVeh), [VehSpd_vVeh]
  [HvCoorn_bHvRlyOpenAct] -> A08_MindChange2ShutHVCal/3(HvCoorn_bHvRlyOpenAct)
  [HvCoorn_bHvRlyOpenAct] -> A10_ShutDisCh2ShutECUCal/2(HvCoorn_bHvRlyOpenAct)
  [HvCoorn_stHVPOld] -> A08_MindChange2ShutHVCal/10(HvCoorn_stHVPOld)
  [HvCoorn_bHvRlyStuck] -> A17_EmergencyShutDownCal/2(HvCoorn_bHvRlyStuck)
  [HvCoorn_bStartUpReq] -> A17_EmergencyShutDownCal/8(HvCoorn_bStartUpReq)
  [HvCoorn_bHvRlyStuck] -> A10_ShutDisCh2ShutECUCal/14(HvCoorn_bHvRlyStuck)
  [HvCoorn_bACChrgLink] -> A22_ModeBMSReqCal/2(HvCoorn_bACChrgLink)
  [HvCoorn_bHvOnFail] -> A10_ShutDisCh2ShutECUCal/8(HvCoorn_bHvOnFail)
  A19_MainProcedure/1(HvCoorn_stHVP) -> A20_HVPStOvrd/1(HvCoorn_stHVPRaw)
  PwrLimBatt_pwrMaxHvesDChrg/1 -> A03_Comm2HVReqCal/1(PwrLimBatt_pwrMaxHvesDChrg), [PwrLimBatt_pwrMaxHvesDChrg]
  [HvCoorn_stHVPOld] -> A17_EmergencyShutDownCal/10(HvCoorn_stHVPOld)
  ved_bHvShtdwn/1 -> A17_EmergencyShutDownCal/11(ved_bHvShtdwn), [ved_bHvShtdwn]
  A17_EmergencyShutDownCal/6(HvCoorn_bEmShutHeal) -> A19_MainProcedure/27(HvCoorn_bEmShutHeal)
  icbms_uHVBat/1 -> A10_ShutDisCh2ShutECUCal/13(icbms_uHVBat)
  [bVolDiffEnaHv] -> A12_ShutECU2CommCal/1(bVolDiffEnaHv)
  icobc_uHvDcAct/1 -> [icobc_uHvDcAct], A17_EmergencyShutDownCal/12(icobc_uHvDcAct)
  icfm_bUActSigErr/1 -> [icfm_bUActSigErr], A17_EmergencyShutDownCal/13(icfm_bUActSigErr)
  icobc_bUHvDcActSigErr/1 -> [icobc_bUHvDcActSigErr], A17_EmergencyShutDownCal/14(icobc_bUHvDcActSigErr)
  icdc_bUHvActSigErr/1 -> [icdc_bUHvActSigErr], A17_EmergencyShutDownCal/15(icdc_bUHvActSigErr)
  [icobc_uHvDcAct] -> A10_ShutDisCh2ShutECUCal/9(icobc_uHvDcAct)
  [icfm_bUActSigErr] -> A10_ShutDisCh2ShutECUCal/10(icfm_bUActSigErr)
  [icobc_bUHvDcActSigErr] -> A10_ShutDisCh2ShutECUCal/11(icobc_bUHvDcActSigErr)
  [icdc_bUHvActSigErr] -> A10_ShutDisCh2ShutECUCal/12(icdc_bUHvActSigErr)
  [HvCoorn_bChrgLink] -> A06_ReadyWait2ReadyCal/3(HvCoorn_bChrgLink)
  [VehSpd_vVeh] -> A24_DCDCModeReqCal/2(VehSpd_vVeh)
  A01_HighvoltPowerUpReq/15(HvCoorn_bRemLvBatMntnReq) -> HvCoorn_bRemLvBatMntnReq/1
  Chrg_stBookChrgMod/1 -> A01_HighvoltPowerUpReq/28(Chrg_stBookChrgMod)
  A01_HighvoltPowerUpReq/6(HvCoorn_bACChrgPause) -> HvCoorn_bACChrgPause/1
  icdc_bStHvilSigErr/1 -> A01_HighvoltPowerUpReq/15(icdc_bStHvilSigErr)
  ian_tAcChrgrNTemp/1 -> A01_HighvoltPowerUpReq/5(ian_tAcChrgrNTemp)
  icacu_stWarmTime/1 -> A01_HighvoltPowerUpReq/6(icacu_stWarmTime)
  icdc_stHvil/1 -> A01_HighvoltPowerUpReq/16(icdc_stHvil)
  icobc_bStAcHvilSigErr/1 -> A01_HighvoltPowerUpReq/20(icobc_bStAcHvilSigErr)
  icbms_stHvil/1 -> A01_HighvoltPowerUpReq/11(icbms_stHvil)
  A01_HighvoltPowerUpReq/5(HvCoorn_bHvilStOk) -> [HvCoorn_bHvilStOk], HvCoorn_bHvilStOk/1
  tcj_bHvBatPrecdngFinish/1 -> A01_HighvoltPowerUpReq/41(tcj_bHvBatPrecdngFinish)
  idi_bHvilInput/1 -> A01_HighvoltPowerUpReq/30(idi_bHvilInput)
  iud_stRemoteImmo/1 -> A01_HighvoltPowerUpReq/34(iud_stRemoteImmo)
  icobc_pwrChrgMax/1 -> A01_HighvoltPowerUpReq/21(icobc_pwrChrgMax)
  A01_HighvoltPowerUpReq/2(HvCoorn_bACChrgLinkOk) -> [HvCoorn_bACChrgLinkOk], HvCoorn_bACChrgLinkOk/1
  A01_HighvoltPowerUpReq/4(HvCoorn_bHvilHwStOk) -> HvCoorn_bHvilHwErr/1
  A01_HighvoltPowerUpReq/8(HvCoorn_bHvRlyOpenAct) -> [HvCoorn_bHvRlyOpenAct], HvCoorn_bHvRlyOpenAct/1
  std_tExterTemp/1 -> A01_HighvoltPowerUpReq/39(std_tExterTemp)
  A01_HighvoltPowerUpReq/7(HvCoorn_bHvRlyClsAct) -> [HvCoorn_bHvRlyClsAct], HvCoorn_bHvRlyClsAct/1
  A01_HighvoltPowerUpReq/12(HvCoorn_bBattWarmReq) -> HvCoorn_bBattWarmReq/1
  icbms_bBatACChrgFull/1 -> A01_HighvoltPowerUpReq/7(icbms_bBatACChrgFull)
  ian_tAcChrgrL1Temp/1 -> A01_HighvoltPowerUpReq/4(ian_tAcChrgrL1Temp)
  A01_HighvoltPowerUpReq/10(HvCoorn_bACLinkTempErr) -> HvCoorn_bACLinkTempErr/1
  ictel_stHvBatPrecdng/1 -> A01_HighvoltPowerUpReq/29(ictel_stHvBatPrecdng)
  icepb_stEpbSys/1 -> A01_HighvoltPowerUpReq/26(icepb_stEpbSys)
  icbms_stMainNegRly/1 -> A01_HighvoltPowerUpReq/12(icbms_stMainNegRly), [icbms_stMainNegRly]
  icbms_stPrecRly/1 -> A01_HighvoltPowerUpReq/14(icbms_stPrecRly)
  A01_HighvoltPowerUpReq/13(HvCoorn_stWarmTimeCfgResp) -> HvCoorn_stWarmTimeCfgResp/1
  iud_bNoHVHWarmTiCfg/1 -> A01_HighvoltPowerUpReq/31(iud_bNoHVHWarmTiCfg)
  A01_HighvoltPowerUpReq/1(HvCoorn_bACChrgLink) -> [HvCoorn_bACChrgLink], HvCoorn_bACChrgLink/1
  A01_HighvoltPowerUpReq/11(HvCoorn_bParked4ChDchg) -> [HvCoorn_bParked4ChDchg], HvCoorn_bParked4ChDchg/1
  icobc_stHvil/1 -> A01_HighvoltPowerUpReq/22(icobc_stHvil)
  iud_stOBCWakeUpOrigin/1 -> A01_HighvoltPowerUpReq/33(iud_stOBCWakeUpOrigin)
  A01_HighvoltPowerUpReq/9(HvCoorn_bHvRlyStuck) -> [HvCoorn_bHvRlyStuck], HvCoorn_bHvRlyStuck/1
  icobc_uChrgrCtrlSigVolt/1 -> A01_HighvoltPowerUpReq/25(icobc_uChrgrCtrlSigVolt)
  iczcu_stRmtChrgReq/1 -> A01_HighvoltPowerUpReq/27(iczcu_stRmtChrgReq)
  icbms_bStHvilSigErr/1 -> A01_HighvoltPowerUpReq/8(icbms_bStHvilSigErr)
  iud_bNoHVHConfig/1 -> A01_HighvoltPowerUpReq/32(iud_bNoHVHConfig)
  A01_HighvoltPowerUpReq/3(HvCoorn_stHvil) -> HvCoorn_stHvil/1
  icbms_stMainPosRly/1 -> [icbms_stMainPosRly], A01_HighvoltPowerUpReq/13(icbms_stMainPosRly)
  A01_HighvoltPowerUpReq/14(HvCoorn_bACChrgEna) -> HvCoorn_bACChrgEna/1
  icobc_bChrgrCtrlSigCnct/1 -> A01_HighvoltPowerUpReq/19(icobc_bChrgrCtrlSigCnct)
  icbms_stHvBat/1 -> [icbms_stHvBat], A01_HighvoltPowerUpReq/10(icbms_stHvBat)
  [icobc_stOBCMode] -> A03_Comm2HVReqCal/9(icobc_stOBCMode)
  [icdc_stMode] -> A03_Comm2HVReqCal/7(icdc_stMode)
  [PwrLimBatt_pwrMaxHvesDChrg] -> A01_HighvoltPowerUpReq/35(PwrLimBatt_pwrMaxHvesDChrg)
  Chrg_bACChrgCmpl/1 -> A01_HighvoltPowerUpReq/36(Chrg_bACChrgCmpl), [Chrg_bACChrgCmpl]
  [idi_bKeyOn] -> A03_Comm2HVReqCal/15(idi_bKeyOn)
  [HvCoorn_bObcChrgrCnct] -> A01_HighvoltPowerUpReq/23(HvCoorn_bObcChrgrCnct)
  [GearLvr_stDrvGear] -> A01_HighvoltPowerUpReq/37(GearLvr_stDrvGear)
  [VehSpd_vVeh] -> A01_HighvoltPowerUpReq/38(VehSpd_vVeh)
  [HvCoorn_bHvilClsReqOld] -> A01_HighvoltPowerUpReq/40(HvCoorn_bHvilClsReqOld)
  [HvCoorn_tiHVPStTimer] -> A03_Comm2HVReqCal/10(HvCoorn_tiHVPStTimer)
  inv_stHvBattWarmTime/1 -> A01_HighvoltPowerUpReq/42(inv_stHvBattWarmTime)
  [icbms_pctHVBatSOCDisp] -> A03_Comm2HVReqCal/4(icbms_pctHVBatSOCDisp)
  icbms_stDcChrgrCnct/1 -> A01_HighvoltPowerUpReq/43(icbms_stDcChrgrCnct), [icbms_stDcChrgrCnct]
  ian_tDcChrgrTemp1/1 -> A01_HighvoltPowerUpReq/44(ian_tDcChrgrTemp1)
  ian_tDcChrgrTemp2/1 -> A01_HighvoltPowerUpReq/45(ian_tDcChrgrTemp2)
  Chrg_bDCChrgCmpl/1 -> A01_HighvoltPowerUpReq/46(Chrg_bDCChrgCmpl), [Chrg_bDCChrgCmpl]
  icbms_bBatDCChrgFull/1 -> A01_HighvoltPowerUpReq/47(icbms_bBatDCChrgFull)
  icbms_uDcChgrCap/1 -> A01_HighvoltPowerUpReq/48(icbms_uDcChgrCap)
  icbms_iDcChgrCap/1 -> A01_HighvoltPowerUpReq/49(icbms_iDcChgrCap)
  icbms_bDcChrgCfg/1 -> A01_HighvoltPowerUpReq/50(icbms_bDcChrgCfg), [icbms_bDcChrgCfg]
  A01_HighvoltPowerUpReq/16(HvCoorn_bDCChrgLink) -> [HvCoorn_bDCChrgLink], HvCoorn_bDCChrgLink/1
  A01_HighvoltPowerUpReq/17(HvCoorn_bChrgLink) -> [HvCoorn_bChrgLink], HvCoorn_bChrgLink/1
  A01_HighvoltPowerUpReq/18(HvCoorn_bDCLinkTempErr) -> HvCoorn_bDCLinkTempErr/1
  A01_HighvoltPowerUpReq/19(HvCoorn_bDCChrgEna) -> HvCoorn_bDCChrgEna/1
  [HvCoorn_tiHVPStTimer] -> A05_DCDCBuck2ReadyCal/1(HvCoorn_tiHVPStTimer)
  [HvCoorn_tiHVPStTimer] -> A08_MindChange2ShutHVCal/2(HvCoorn_tiHVPStTimer)
  [HvCoorn_tiHVPStTimer] -> A10_ShutDisCh2ShutECUCal/1(HvCoorn_tiHVPStTimer)
  [HvCoorn_tiHVPStTimer] -> A11_ShutECU2AftRunCal/1(HvCoorn_tiHVPStTimer)
  [HvCoorn_tiHVPStTimer] -> A13_AftRun2NetManCal/1(HvCoorn_tiHVPTimer)
  [HvCoorn_tiHVPStTimer] -> A15_Wake2NetManCal/2(HvCoorn_tiHVPTimer)
  [HvCoorn_tiHVPStTimer] -> A16_Init2AftRunCal/2(HvCoorn_tiHVPTimer), A17_EmergencyShutDownCal/1(HvCoorn_tiHVPStTimer)
  A02_Init2StupCal/1(HvCoorn_tiHVPStTimer) -> [HvCoorn_tiHVPStTimer]
  [icbms_stHvBat] -> A03_Comm2HVReqCal/6(icbms_stHvBat)
  [icfm_stMode] -> A03_Comm2HVReqCal/8(icfm_stMode)
  [HvCoorn_bDCChrgLink] -> A03_Comm2HVReqCal/16(HvCoorn_bDCChrgLink)
  A09_ShutHV2ShutDisChCal/1(HvCoorn_bShutHV2ShutDisCh) -> A19_MainProcedure/13(HvCoorn_bShutHV2ShutDisCh)
  [icbms_bDcChrgCfg] -> A22_ModeBMSReqCal/6(icbms_bDcChrgCfg)
  [Chrg_bDCChrgCmpl] -> A22_ModeBMSReqCal/7(Chrg_bDCChrgCmpl)
  A22_ModeBMSReqCal/3(HvCoorn_bHvReady) -> [HvCoorn_bHvReady], HvCoorn_bHvReady/1
  Unit Delay3/1 -> [HvCoorn_bHvilClsReqOld]
  A23_MCUModeReqCal/2(HvCoorn_stRMCUModeReq) -> HvCoorn_stRMCUModeReq/1
  icrm_nAct/1 -> [icrm_nAct], A17_EmergencyShutDownCal/16(icrm_nAct)
  icrm_uAct/1 -> [icrm_uAct], A17_EmergencyShutDownCal/18(icrm_uAct)
  [icrm_uAct] -> A04_HVReq2DCBuckCal/11(icrm_uAct)
  icrm_bUActSigErr/1 -> [icrm_bUActSigErr], A17_EmergencyShutDownCal/17(icrm_bUActSigErr)
  [icrm_bUActSigErr] -> A10_ShutDisCh2ShutECUCal/16(icrm_bUActSigErr)
  [icrm_nAct] -> A09_ShutHV2ShutDisChCal/3(icrm_nAct)
  icrm_stMode/1 -> [icrm_stMode], A01_HighvoltPowerUpReq/51(icrm_stMode)
  [icrm_stMode] -> A03_Comm2HVReqCal/17(icrm_stMode)
  [icrm_stMode] -> A04_HVReq2DCBuckCal/12(icrm_stMode)
  [icrm_stMode] -> A07_MindChange2ReadyCal/4(icrm_stMode)
  [icrm_stMode] -> A08_MindChange2ShutHVCal/5(icrm_stMode)
  [icrm_stMode] -> A10_ShutDisCh2ShutECUCal/6(icrm_stMode)
  [icrm_stMode] -> A17_EmergencyShutDownCal/19(icrm_stMode)
  [icrm_uAct] -> A10_ShutDisCh2ShutECUCal/15(icrm_uAct)
  [icrm_uAct] -> A11_ShutECU2AftRunCal/5(icrm_uAct)
  VehCfg_bFrntMotByp/1 -> A01_HighvoltPowerUpReq/52(VehCfg_bFrntMotByp), [VehCfg_bFrntMotByp]
  [VehCfg_bFrntMotByp] -> A08_MindChange2ShutHVCal/12(VehCfg_bFrntMotByp)
  [VehCfg_bFrntMotByp] -> A10_ShutDisCh2ShutECUCal/17(VehCfg_bFrntMotByp)
  [VehCfg_bFrntMotByp] -> A23_MCUModeReqCal/2(VehCfg_bFrntMotByp)
  [idi_bKeyStrt] -> A01_HighvoltPowerUpReq/53(idi_bKeyStrt)
  icfm_stActvDchrg/1 -> A10_ShutDisCh2ShutECUCal/18(icfm_stActvDchrg)
  icrm_stActvDchrg/1 -> A10_ShutDisCh2ShutECUCal/19(icrm_stActvDchrg)
  A10_ShutDisCh2ShutECUCal/4(HvCoorn_bMCUActvDchrgCmpl) -> [HvCoorn_bMCUActvDchrgCmpl]
  A10_ShutDisCh2ShutECUCal/5(HvCoorn_bMCUActvDchrgErr) -> [HvCoorn_bMCUActvDchrgErr]
  [HvCoorn_bMCUActvDchrgCmpl] -> A17_EmergencyShutDownCal/20(HvCoorn_bMCUActvDchrgCmpl)
  [HvCoorn_bMCUActvDchrgErr] -> A17_EmergencyShutDownCal/21(HvCoorn_bMCUActvDchrgErr)
  A22_ModeBMSReqCal/4(HvCoorn_bDrvRdy) -> HvCoorn_bDrvRdy/1
  [GearLvr_stDrvGear] -> A22_ModeBMSReqCal/8(GearLvr_stDrvGear)
  BrkPedDev_bBrk/1 -> [BrkPedDev_bBrk], A06_ReadyWait2ReadyCal/6(BrkPedDev_bBrk)
  icbms_bDcChrgWkup/1 -> A01_HighvoltPowerUpReq/54(icbms_bDcChrgWkup)
  [HvCoorn_bHvReady] -> A01_HighvoltPowerUpReq/1(HvCoorn_bHvReady)
  [BrkPedDev_bBrk] -> A01_HighvoltPowerUpReq/2(BrkPedDev_bBrk)
  Chrg_bChrgErrForever/1 -> A01_HighvoltPowerUpReq/55(Chrg_bChrgErrForever)
  icbms_stDcChrg/1 -> A04_HVReq2DCBuckCal/13(icbms_stDcChrg)
  [icbms_stDcChrgrCnct] -> A04_HVReq2DCBuckCal/14(icbms_stDcChrgrCnct)
  [HvCoorn_stHVPOld] -> A05_DCDCBuck2ReadyCal/4(HvCoorn_stHVPOld)
  A05_DCDCBuck2ReadyCal/2(HvCoorn_bDCBuck2Shtdwn) -> A19_MainProcedure/8(HvCoorn_bDCBuck2Shtdwn)
  [icbms_stHvBat] -> A23_MCUModeReqCal/3(icbms_stHvBat)
  [VehSpd_vVeh] -> A23_MCUModeReqCal/4(VehSpd_vVeh)
  [GearLvr_stDrvGear] -> A23_MCUModeReqCal/5(GearLvr_stDrvGear)
  icecc_bStalHeatReq/1 -> A23_MCUModeReqCal/6(icecc_bStalHeatReq)
  icrm_stPlsHeatg/1 -> A23_MCUModeReqCal/7(icrm_stPlsHeatg)
  A23_MCUModeReqCal/3(HvCoorn_bRMCUPlsHeatgReq) -> HvCoorn_bRMCUPlsHeatgReq/1
  [HvCoorn_bChrgLink] -> A23_MCUModeReqCal/8(HvCoorn_bChrgLink)
  icrm_stStalHeatg/1 -> A23_MCUModeReqCal/9(icrm_stStalHeatg)
  A23_MCUModeReqCal/4(HvCoorn_bRMCUStalHeatgReq) -> HvCoorn_bRMCUStalHeatgReq/1
  icbms_bHvShutOffReq/1 -> A01_HighvoltPowerUpReq/56(icbms_bHvShutOffReq)
  iczcu_bHVPwrOffReq/1 -> A01_HighvoltPowerUpReq/57(iczcu_bHVPwrOffReq)
  icbms_bPlsHeatReq/1 -> A23_MCUModeReqCal/10(icbms_bPlsHeatReq)
  icecc_bHVReq/1 -> A01_HighvoltPowerUpReq/58(icecc_bHVReq)
  A22_ModeBMSReqCal/5(HvCoorn_bEccEna) -> HvCoorn_bEccEna/1
  [HvCoorn_stHVPOld] -> A01_HighvoltPowerUpReq/59(HvCoorn_stHVPOld)
  A08_MindChange2ShutHVCal/2(HvCoorn_bVehSpd4HvDown) -> A19_MainProcedure/29(HvCoorn_bVehSpd4HvDown)
  [HvCoorn_bHvRlyOpenAct] -> A27_ErrCheck/5(HvCoorn_bHvRlyOpenAct)
  icbms_uDCLnk/1 -> A27_ErrCheck/4(icbms_uDCLnk)
  [icfm_uAct] -> A27_ErrCheck/7(icfm_uAct)
  [icrm_uAct] -> A27_ErrCheck/6(icrm_uAct)
  icbms_stPrechrgMod/1 -> A27_ErrCheck/3(icbms_stPrechrgMod)
  DTC_bDiagRst/1 -> [DTC_bDiagRst], A27_ErrCheck/2(DTC_bDiagRst)
  A27_ErrCheck/1(HvCoorn_bHvRlyUnexpdDcnctErr) -> HvCoorn_bHvRlyUnexpdDcnctErr/1
  A27_ErrCheck/2(HvCoorn_bBMSUnexpdDcnctErr) -> HvCoorn_bBMSUnexpdDcnctErr/1
  A27_ErrCheck/3(HvCoorn_bMainRlyFail2ClsErr) -> HvCoorn_bMainRlyFail2ClsErr/1
  A27_ErrCheck/4(HvCoorn_bPrechrgOvtiErr) -> HvCoorn_bPrechrgOvtiErr/1
  A27_ErrCheck/5(HvCoorn_bDchrgOvtiErr) -> HvCoorn_bDchrgOvtiErr/1
  DTC_bDiagEnaCdnWkupLong/1 -> A27_ErrCheck/11(DTC_bDiagEnaCdnWkupLong)
  ipf_bPCAN0x130Vld/1 -> A27_ErrCheck/12(ipf_bPCAN0x130Vld), [ipf_bPCAN0x130Vld]
  ipf_bPCAN0x111S1Vld/1 -> A27_ErrCheck/13(ipf_bPCAN0x111S1Vld), [ipf_bPCAN0x111S1Vld]
  ipf_bPCAN0x110S1Vld/1 -> A27_ErrCheck/14(ipf_bPCAN0x110S1Vld)
  ipf_bPCANBusOffErr/1 -> A27_ErrCheck/15(ipf_bPCANBusOffErr)
  [HvCoorn_bCtrlrHvilErr] -> A27_ErrCheck/10(HvCoorn_bCtrlrHvilErr)
  A27_ErrCheck/7(HvCoorn_bBMSHvilErr) -> HvCoorn_bBMSHvilErr/1
  icecc_bWPTCHvilFlt/1 -> A01_HighvoltPowerUpReq/60(icecc_bWPTCHvilFlt)
  icecc_bEASHvilFlt/1 -> A01_HighvoltPowerUpReq/61(icecc_bEASHvilFlt)
  [ipf_bPCAN0x130Vld] -> A03_Comm2HVReqCal/18(ipf_bPCAN0x130Vld)
  [ipf_bPCAN0x111S1Vld] -> A03_Comm2HVReqCal/19(ipf_bPCAN0x111S1Vld)
  DTC_bDiagEnaCdnWkupSho/1 -> A27_ErrCheck/16(DTC_bDiagEnaCdnWkupSho), [DTC_bDiagEnaCdnWkupSho]
  [DTC_bDiagEnaCdnWkupSho] -> A03_Comm2HVReqCal/20(DTC_bDiagEnaCdnWkupSho)
  ipf_bPCAN0x353Vld/1 -> A27_ErrCheck/8(ipf_bPCAN0x353Vld)
  [icdc_uHvAct] -> A27_ErrCheck/9(icdc_uHvAct)
  A27_ErrCheck/6(HvCoorn_bDCUnexpdDcnctErr) -> HvCoorn_bDCUnexpdDcnctErr/1
  iczcu_stFMCUAuthent/1 -> A06_ReadyWait2ReadyCal/7(iczcu_stFMCUAuthent)
  DrvMod_bVehShowMod/1 -> [DrvMod_bVehShowMod], A06_ReadyWait2ReadyCal/8(DrvMod_bVehShowMod)
  icicm_bPwrOffReq/1 -> A01_HighvoltPowerUpReq/62(icicm_bPwrOffReq)
  icisg_nAct/1 -> A09_ShutHV2ShutDisChCal/4(icisg_nAct)
  A23_MCUModeReqCal/5(HvCoorn_stISGModeReq) -> HvCoorn_stISGModeReq/1
  ved_bInhbHvOn/1 -> A01_HighvoltPowerUpReq/73(ved_bInhbHvOn)
  ved_bInhbRdy/1 -> A06_ReadyWait2ReadyCal/9(ved_bInhbRdy)
  ved_bEmgcyHvShtdwn/1 -> A18_ShutDownReqCal/1(ved_bEmgcyHvShtdwn)
  [ved_bHvShtdwn] -> A01_HighvoltPowerUpReq/63(ved_bHvShtdwn)
  ipf_bBD1CAN0x41CVld/1 -> A01_HighvoltPowerUpReq/64(ipf_bBD1CAN0x41CVld)
  icbms_stIsolTst/1 -> A06_ReadyWait2ReadyCal/10(icbms_stIsolTst)
  icicm_bOTAOn/1 -> [icicm_bOTAOn], A01_HighvoltPowerUpReq/65(icicm_bOTAOn)
  icicm_stHVReq/1 -> A01_HighvoltPowerUpReq/66(icicm_stHVReq)
  [icicm_bOTAOn] -> A06_ReadyWait2ReadyCal/11(icicm_bOTAOn)
  icobc_bDchrgrCnct/1 -> A01_HighvoltPowerUpReq/67(icobc_bDchrgrCnct), [icobc_bDchrgrCnct]
  A01_HighvoltPowerUpReq/20(HvCoorn_stStartUpReq) -> [HvCoorn_stStartUpReq], HvCoorn_stStartUpReq/1
  ictcp_stRmtHvReq/1 -> A01_HighvoltPowerUpReq/68(ictcp_stRmtHvReq)
  [HvCoorn_bParked4ChDchg] -> A28_V2L/5(HvCoorn_bParked4ChDchg)
  [icobc_bDchrgrCnct] -> A28_V2L/4(icobc_bDchrgrCnct)
  icbms_pctHVBatSOCDisp/1 -> A28_V2L/6(icbms_pctHVBatSOCDisp), [icbms_pctHVBatSOCDisp]
  icicm_pctSOCV2XLimSet/1 -> A28_V2L/7(icicm_pctSOCV2XLimSet)
  [icobc_stOBCMode] -> A28_V2L/8(icobc_stOBCMode)
  icicm_stIvtrSwt/1 -> A28_V2L/2(icicm_stIvtrSwt)
  [HvCoorn_bDCChrgLink] -> A28_V2L/9(HvCoorn_bDCChrgLink)
  A28_V2L/1(HvCoorn_bV2LReq) -> HvCoorn_bV2LReq/1
  A28_V2L/2(HvCoorn_bV2LActv) -> [HvCoorn_bV2LActv], HvCoorn_bV2LActv/1
  A21_ShutDwnEna/1(HvCoorn_bAllwShutNet) -> HvCoorn_bAllwShutNet/1
  A21_ShutDwnEna/2(HvCoorn_bAllwSlep) -> HvCoorn_bAllwSlep/1
  iczcu_stCarMod/1 -> A01_HighvoltPowerUpReq/69(iczcu_stCarMod)
  [HvCoorn_bV2LActv] -> Unit Delay4/1
  Unit Delay4/1 -> A01_HighvoltPowerUpReq/70(HvCoorn_bV2LActv)
  ParkCtrl_bRPAActv/1 -> A06_ReadyWait2ReadyCal/12(ParkCtrl_bRPAActv)
  icbms_stChrgSts/1 -> A27_ErrCheck/17(icbms_stChrgSts)
  ipf_bPCAN0x343S2Vld/1 -> A27_ErrCheck/18(ipf_bPCAN0x343S2Vld)
  [DTC_bDiagRst] -> A03_Comm2HVReqCal/21(DTC_bDiagRst)
  HvCoorn_pctSOCV2XLimSetEER/1 -> A28_V2L/10(HvCoorn_pctSOCV2XLimSetEER)
  A28_V2L/3(HvCoorn_pctSOCV2XLimSetEEW) -> HvCoorn_pctSOCV2XLimSetEEW/1
  [HvCoorn_stStartUpReq] -> A04_HVReq2DCBuckCal/15(HvCoorn_stStartUpReq)
  [HvCoorn_stHVPOld] -> A06_ReadyWait2ReadyCal/13(HvCoorn_stHVPOld)
  A04_HVReq2DCBuckCal/4(HvCoorn_bHvOnFailRst) -> [HvCoorn_bHvOnFailRst]
  [HvCoorn_bHvInitFail] -> A01_HighvoltPowerUpReq/71(HvCoorn_bHvInitFail)
  [HvCoorn_bHvOnFail] -> A01_HighvoltPowerUpReq/72(HvCoorn_bHvOnFai)
  [HvCoorn_bHvOnFailRst] -> A03_Comm2HVReqCal/22(HvCoorn_bHvOnFailRst)
  Chrg_bChrgStopBySOCLim/1 -> A01_HighvoltPowerUpReq/74(Chrg_bChrgStopBySOCLim)
  Chrg_bBookChrgCmpl/1 -> A01_HighvoltPowerUpReq/75(Chrg_bBookChrgCmpl)
  iud_bNetMaintn/1 -> A14_NetMan2PwrShutCal/1(VCCM_bNetMaintn)
  [HvCoorn_bHvOnFail] -> A27_ErrCheck/19(HvCoorn_bHvOnFail)
  [icfm_uAct] -> A07_MindChange2ReadyCal/5(icfm_uAct)
  [icrm_uAct] -> A07_MindChange2ReadyCal/6(icrm_uAct)
  icobc_bVehCnct/1 -> A01_HighvoltPowerUpReq/76(icobc_bVehCnct)
  A06_ReadyWait2ReadyCal/3(HvCoorn_stRdy2RdyWait) -> HvCoorn_stRdy2RdyWait/1
  A06_ReadyWait2ReadyCal/4(HvCoorn_bAuthentPass) -> HvCoorn_bAuthentPass/1
  icobc_stChrgrCnct/1 -> [icobc_stChrgrCnct], A04_HVReq2DCBuckCal/7(icobc_stChrgrCnct)
  icisg_uAct/1 -> [icisg_uAct], A04_HVReq2DCBuckCal/16(icisg_uAct)
  [icisg_uAct] -> A10_ShutDisCh2ShutECUCal/20(icisg_uAct)
  icisg_stMod/1 -> [icisg_stMod], A08_MindChange2ShutHVCal/13(icisg_stMod)
  A04_HVReq2DCBuckCal/5(HvCoorn_bObcChrgrCnct) -> [HvCoorn_bObcChrgrCnct]
  [VehCfg_bFrntMotByp] -> A04_HVReq2DCBuckCal/17(VehCfg_bFrntMotByp)
  [icicm_bOTAOn] -> A28_V2L/11(icicm_bOTAOn)
  [icbms_pctHVBatSOCDisp] -> A01_HighvoltPowerUpReq/9(icbms_pctHVBatSOCDisp)
  [HvCoorn_tiHVPStTimer] -> A09_ShutHV2ShutDisChCal/5(HvCoorn_tiHVPStTimer)
  [HvCoorn_stHVPOld] -> A09_ShutHV2ShutDisChCal/6(HvCoorn_stHVPOld)
  icdkm_stLrcpReq/1 -> A06_ReadyWait2ReadyCal/14(icdkm_stLrcpReq)
  ictcp_stLostComWarn/1 -> A06_ReadyWait2ReadyCal/15(ictcp_stLostComWarn)
  [HvCoorn_tiHVPStTimer] -> A14_NetMan2PwrShutCal/2(HvCoorn_tiHVPStTimer)
  [HvCoorn_stHVPOld] -> A14_NetMan2PwrShutCal/3(HvCoorn_stHVPOld)
  A01_HighvoltPowerUpReq/21(HvCoorn_bCtrlrHvilErr) -> [HvCoorn_bCtrlrHvilErr]
  A27_ErrCheck/8(HvCoorn_bFMCUHvilErr) -> HvCoorn_bFMCUHvilErr/1
  A27_ErrCheck/9(HvCoorn_bRMCUHvilErr) -> HvCoorn_bRMCUHvilErr/1
  A27_ErrCheck/10(HvCoorn_bOBCHvilErr) -> HvCoorn_bOBCHvilErr/1
  A27_ErrCheck/11(HvCoorn_bDCDCHvilErr) -> HvCoorn_bDCDCHvilErr/1
  A27_ErrCheck/12(HvCoorn_bHWHvilErr) -> HvCoorn_bHWHvilErr/1
  A27_ErrCheck/13(HvCoorn_bWPTCHvilErr) -> HvCoorn_bWPTCHvilErr/1
  A27_ErrCheck/14(HvCoorn_bEASHvilErr) -> HvCoorn_bEASHvilErr/1
  iczcu_stRMCUAuthent/1 -> A06_ReadyWait2ReadyCal/16(iczcu_stRMCUAuthent)
  [VehCfg_bFrntMotByp] -> A06_ReadyWait2ReadyCal/17(VehCfg_bFrntMotByp)
  icfm_bHvilFlt/1 -> A01_HighvoltPowerUpReq/77(icfm_bHvilFlt)
  icrm_bHvilFlt/1 -> A01_HighvoltPowerUpReq/78(icrm_bHvilFlt)
  A06_ReadyWait2ReadyCal/5(HvCoorn_bMCUAuthentPass) -> HvCoorn_bMCUAuthentPass/1
  PwrLimBatt_pwrContnsDChrg/1 -> [PwrLimBatt_pwrContnsDChrg], A29_V2In/3(PwrLimBatt_pwrContnsDChrg)
  [idi_bKeyOn] -> A29_V2In/1(idi_bKeyOn)
  A20_HVPStOvrd/1(HvCoorn_stHVP) -> A29_V2In/2(HvCoorn_stHVP), A28_V2L/1(HvCoorn_stHVP), [HvCoorn_stHVP], HvCoorn_stHVP/1, Unit Delay2/1, A21_ShutDwnEna/1(HvCoorn_stHVP), A22_ModeBMSReqCal/1(HvCoorn_stHVP), A23_MCUModeReqCal/1(HvCoorn_stHVP), A24_DCDCModeReqCal/1(HvCoorn_stHVP), A25_HvilClsReqCal/1(HvCoorn_stHVP), A26_DischargeErrCal/1(HvCoorn_stHVP), A27_ErrCheck/1(HvCoorn_stHVP)
  [ved_bHvShtdwn] -> A29_V2In/9(ved_bHvShtdwn)
  [icobc_stChrgrCnct] -> A29_V2In/6(icobc_stChrgrCnct)
  [icbms_pctHVBatSOCDisp] -> A29_V2In/4(icbms_pctHVBatSOCDisp)
  ibsw_bCnctElecDvce/1 -> A29_V2In/8(ibsw_bCnctElecDvce)
  A29_V2In/1(HvCoorn_bV2InReq) -> HvCoorn_bV2InReq/1
  icicm_stIvtrEnaSwt/1 -> A29_V2In/7(icicm_stIvtrEnaSwt)
  A29_V2In/2(HvCoorn_bV2InEna) -> HvCoorn_bV2InEna/1
  icbms_bIsolFlt/1 -> A27_ErrCheck/21(icbms_bIsolFlt)
  ipf_bPCAN0x340S1Vld/1 -> A27_ErrCheck/20(ipf_bPCAN0x340S1Vld)
  A27_ErrCheck/15(HvCoorn_bBMSIsoErr) -> HvCoorn_bBMSIsoErr/1
  [HvCoorn_stHVPOld] -> A30_ISGNotRdy/3(HvCoorn_stHVPOld)
  icems_stEng/1 -> [icems_stEng], A30_ISGNotRdy/2(icems_stEng)
  [HvCoorn_bStartUpReq] -> A30_ISGNotRdy/1(HvCoorn_bStartUpReq)
  A30_ISGNotRdy/1(HvCoorn_bAPUNotRdy) -> A19_MainProcedure/30(HvCoorn_bAPUNotRdy)
  GearLvr_bNapModActv/1 -> A06_ReadyWait2ReadyCal/18(GearLvr_bNapModActv)
  GearLvr_stCmpgMod/1 -> A06_ReadyWait2ReadyCal/19(GearLvr_stCmpgMod)
  GearLvr_bOffVehPwrKeep/1 -> A06_ReadyWait2ReadyCal/20(GearLvr_bOffVehPwrKeep)
  GearLvr_bSentilMod/1 -> A06_ReadyWait2ReadyCal/21(GearLvr_bSentilMod)
  A01_HighvoltPowerUpReq/22(HvCoorn_bKeyOnPwrUp) -> HvCoorn_bKeyOnPwrUp/1
  icbms_tMaxBat/1 -> A01_HighvoltPowerUpReq/80(icbms_tMaxBat)
  icbms_tMinBat/1 -> A01_HighvoltPowerUpReq/81(icbms_tMinBat)
  icebs_tLvBat/1 -> A01_HighvoltPowerUpReq/82(icebs_tLvBat)
  icebs_pctLvBatSoc/1 -> A01_HighvoltPowerUpReq/83(icebs_pctLvBatSoc)
  icebs_pctLvBatSoh/1 -> A01_HighvoltPowerUpReq/79(icebs_pctLvBatSoh)
  icebs_stSocPrcsn/1 -> A01_HighvoltPowerUpReq/84(icebs_stSocPrcsn)
  icebs_uLvBat/1 -> A01_HighvoltPowerUpReq/85(icebs_uLvBat)
  icicm_stOTAPwrMngtReq/1 -> A01_HighvoltPowerUpReq/86(icicm_stOTAPwrMngtReq)
  HvCoorn_ctSmtBatMntnFailEER/1 -> A01_HighvoltPowerUpReq/87(HvCoorn_ctSmtBatMntnFailEER)
  iud_bEEIniFnsd/1 -> A01_HighvoltPowerUpReq/88(iud_bEEIniFnsd)
  A01_HighvoltPowerUpReq/23(HvCoorn_bSocWkup) -> HvCoorn_bSocWkup/1
  A01_HighvoltPowerUpReq/24(HvCoorn_ctSmtBatMntnFailEEW) -> HvCoorn_ctSmtBatMntnFailEEW/1
  A01_HighvoltPowerUpReq/25(HvCoorn_stRemLvBatMntnFailRsn) -> HvCoorn_stRemLvBatMntnFailRsn/1
  A01_HighvoltPowerUpReq/26(HvCoorn_ctSmtBatMntnSucsEEW) -> HvCoorn_ctSmtBatMntnSucsEEW/1
  HvCoorn_ctSmtBatMntnSucsEER/1 -> A01_HighvoltPowerUpReq/89(HvCoorn_ctSmtBatMntnSucsEER)
  A01_HighvoltPowerUpReq/27(HvCoorn_bTimerWkupReq) -> HvCoorn_bTimerWkupReq/1
  A01_HighvoltPowerUpReq/30(HvCoorn_bLbmsSocWkup) -> HvCoorn_bLbmsSocWkup/1
  A01_HighvoltPowerUpReq/29(HvCoorn_pctLbmsSocMntnThd) -> HvCoorn_pctLbmsSocMntnThd/1
  A01_HighvoltPowerUpReq/28(HvCoorn_bLbmsLvBatMntnReq) -> HvCoorn_bLbmsLvBatMntnReq/1
  iclbms_stLvRemChrgReq/1 -> A01_HighvoltPowerUpReq/90(iclbms_stLvRemChrgReq)
  ipf_bLBMSCANVld/1 -> A01_HighvoltPowerUpReq/91(ipf_bLBMSCANVld)
  VehCfg_stLvBattTyp/1 -> A01_HighvoltPowerUpReq/92(VehCfg_stLvBattTyp)
  icems_nAct/1 -> [icems_nAct], A30_ISGNotRdy/4(icems_nAct)
  EngStrtStop_bFuChrgActvEEW/1 -> A28_V2L/12(EngStrtStop_bFuChrgActvEEW)
  [icisg_uAct] -> A07_MindChange2ReadyCal/7(icisg_uAct)
  [icobc_stOBCMode] -> A29_V2In/10(icobc_stOBCMode)
  icobc_stOBCModeV2In/1 -> A29_V2In/5(icobc_stOBCModeV2In)
  icisg_bHvilFlt/1 -> A01_HighvoltPowerUpReq/93(icisg_bHvilFlt)
  A27_ErrCheck/16(HvCoorn_bISGHvilErr) -> HvCoorn_bISGHvilErr/1
  A30_Authcation/12(HvCoorn_stTboxByte4Req) -> Terminator7/1
  A30_Authcation/11(HvCoorn_stTboxByte5Req) -> Terminator6/1
  VCCM_flg_Antitheft_Overtime/1 -> A30_Authcation/4(VCCM_flg_Antitheft_Overtime)
  VCCM_flg_Antitheft_Start/1 -> A30_Authcation/5(VCCM_flg_Antitheft_Start)
  A30_Authcation/14(HvCoorn_stVcuByte2Fb) -> Terminator9/1
  A30_Authcation/18(HvCoorn_noVcuAuthReq) -> HvCoorn_noVcuAuthReq/1
  [HvCoorn_stHVPOld] -> A30_Authcation/8(HvCoorn_stHVPOld)
  A30_Authcation/7(HvCoorn_stVcuByte4Req) -> Terminator5/1
  A30_Authcation/16(HvCoorn_stVcuByte0Fb) -> Terminator11/1
  A30_Authcation/8(HvCoorn_bAuthHvStrtLim) -> [HvCoorn_bAuthHvStrtLim]
  ictcp_noAuthSts/1 -> A30_Authcation/7(ictcp_noAuthSts)
  A30_Authcation/9(HvCoorn_bClearZero) -> Terminator12/1
  A30_Authcation/20(" HvCoorn_bAuthFailSpdLim") -> HvCoorn_bAuthFailSpdLim/1
  ictcp_noAuthChlgOnReq/1 -> A30_Authcation/6(ictcp_noAuthChlgOnReq)
  A30_Authcation/13(HvCoorn_stVcuByte3Fb) -> Terminator8/1
  A30_Authcation/2(HvCoorn_bAntiTrig430) -> HvCoorn_bAntiTrig430/1
  A30_Authcation/19(HvCoorn_stVcuByte7Fb) -> Terminator13/1
  A30_Authcation/3(HvCoorn_bAntiTrig42C) -> HvCoorn_bAntiTrig42C/1
  VCCM_flg_Allow_Antitheft/1 -> A30_Authcation/3(VCCM_flg_Allow_Antitheft)
  A30_Authcation/15(HvCoorn_stVcuByte1Fb) -> Terminator10/1
  A30_Authcation/10(HvCoorn_stAuthChkFailLvl) -> HvCoorn_stAuthChkFailLvl/1
  VCU_E2_counterfaieldEER/1 -> A30_Authcation/1(VCU_E2_counterfaieldEER)
  A30_Authcation/6(HvCoorn_stVcuByte5Req) -> Terminator4/1
  A30_Authcation/5(HvCoorn_authfailed_conter) -> Terminator3/1
  A30_Authcation/17(HvCoorn_noVcuAuthFb) -> HvCoorn_noVcuAuthFb/1
  A30_Authcation/1(VCU_Instruction_Type_FB) -> Terminator2/1
  A30_Authcation/4(VCU_E2_counterfaieldEEW) -> VCU_E2_counterfaieldEEW/1
  VCCM_flg_SK_Recep_ok/1 -> A30_Authcation/9(VCCM_flg_SK_Recep_ok)
  [idi_bKeyOn] -> A30_Authcation/2(idi_bKeyOn)
  [HvCoorn_bAuthHvStrtLim] -> A06_ReadyWait2ReadyCal/22(HvCoorn_bAuthHvStrtLim)
  idi_uPwrSply/1 -> A01_HighvoltPowerUpReq/94(idi_uPwrSply)
  A01_HighvoltPowerUpReq/31(HvCoorn_bVehNetWkupEna) -> HvCoorn_bVehNetWkupEna/1
  EngStrtStop_bHVPRdy/1 -> A31_VoltModReq/1(EngStrtStop_bHVPRdy)
  A31_VoltModReq/1(HvCoorn_bDft2EngStrt) -> A32_VoltModSts/1(HvCoorn_bDft2EngStrt)
  A31_VoltModReq/2(HvCoorn_bEngStrt2HvDisb) -> A32_VoltModSts/2(HvCoorn_bEngStrt2HvDisb)
  A31_VoltModReq/3(HvCoorn_bHvDisb2HvDcnct) -> A32_VoltModSts/3(HvCoorn_bHvDisb2HvDcnct)
  A31_VoltModReq/4(HvCoorn_bHvDcnct2HvReq) -> A32_VoltModSts/4(HvCoorn_bHvDcnct2HvReq)
  A31_VoltModReq/5(HvCoorn_bHvReq2VoltModRdy) -> A32_VoltModSts/5(HvCoorn_bHvReq2VoltModRdy)
  A32_VoltModSts/1(HvCoorn_stVoltMod) -> UnitDelay/1, [HvCoorn_stVoltMod], HvCoorn_stVoltMod/1
  UnitDelay/1 -> [HvCoorn_stVoltModOld]
  A32_VoltModSts/2(HvCoorn_bVoltModStbReq) -> HvCoorn_bVoltModStbReq/1, [HvCoorn_bVoltModStbReq]
  DTC_bBMSFltLvl6/1 -> [DTC_bBMSFltLvl6], A31_VoltModReq/3(DTC_bBMSFltLvl6)
  DTC_bBMSFltLvl7/1 -> A31_VoltModReq/4(DTC_bBMSFltLvl7)
  DTC_bBMSFltLvl8/1 -> A31_VoltModReq/5(DTC_bBMSFltLvl8)
  [HvCoorn_stVoltModOld] -> A31_VoltModReq/6(HvCoorn_stVoltModOld)
  EngStrtStop_bEngStrtAllw/1 -> A31_VoltModReq/7(EngStrtStop_bEngStrtAllw)
  HybCoorn_bEngStrtFail/1 -> A31_VoltModReq/8(HybCoorn_bEngStrtFail)
  ved_bInhbEngStrt/1 -> [ved_bInhbEngStrt], A31_VoltModReq/10(ved_bInhbEngStrt)
  [ipf_bPCAN0x130Vld] -> A31_VoltModReq/2(ipf_bPCAN0x130Vld)
  [icems_stEng] -> A31_VoltModReq/9(icems_stEng)
  [icems_nAct] -> A31_VoltModReq/11(icems_nAct)
  [icbms_stMainPosRly] -> A31_VoltModReq/12(icbms_stMainPosRly)
  [icbms_stMainNegRly] -> A31_VoltModReq/13(icbms_stMainNegRly)
  [icbms_iHVBat] -> A31_VoltModReq/14(icbms_iHVBat)
  [icfm_uAct] -> A31_VoltModReq/15(icfm_uAct)
  [icdc_uHvAct] -> A31_VoltModReq/16(icdc_uHvAct)
  [icisg_uAct] -> A31_VoltModReq/17(icisg_uAct)
  [icisg_stMod] -> A31_VoltModReq/18(icisg_stMod)
  [icfm_uAct] -> A33_ISGVoltReq/1(icfm_uAct)
  [icdc_uHvAct] -> A33_ISGVoltReq/2(icdc_uHvAct)
  [icisg_uAct] -> A33_ISGVoltReq/3(icisg_uAct)
  [HvCoorn_stVoltMod] -> A33_ISGVoltReq/4(HvCoorn_stVoltMod)
  A31_VoltModReq/20(HvCoorn_bVoltModHvDisbOvtiErr) -> HvCoorn_bVoltModHvDisbOvtiErr/1
  A31_VoltModReq/21(HvCoorn_bVoltModHvDcnctOvtiErr) -> HvCoorn_bVoltModHvDcnctOvtiErr/1
  A31_VoltModReq/22(HvCoorn_bVoltModHvReqOvtiErr) -> HvCoorn_bVoltModHvReqOvtiErr/1
  A33_ISGVoltReq/1(HvCoorn_uISGReq) -> HvCoorn_uISGReq/1
  [HvCoorn_bVoltModStbReq] -> A22_ModeBMSReqCal/9(HvCoorn_bVoltModStbReq)
  [HvCoorn_stVoltMod] -> A22_ModeBMSReqCal/10(HvCoorn_stVoltMod)
  [HvCoorn_bVoltModStbReq] -> A23_MCUModeReqCal/11(HvCoorn_bVoltModStbReq)
  [HvCoorn_bVoltModStbReq] -> A24_DCDCModeReqCal/3(HvCoorn_bVoltModStbReq)
  ipf_bLIN9EBS0x34NodLostErr/1 -> A01_HighvoltPowerUpReq/95(ipf_bLIN9EBS0x34NodLostErr)
  HvGrid_pwrMotDChrgMax/1 -> Terminator/1
  [PwrLimBatt_pwrContnsDChrg] -> A28_V2L/3(PwrLimBatt_pwrContnsDChrg)
  DTC_bBMSFltLvl5/1 -> A31_VoltModReq/19(DTC_bBMSFltLvl5)
  EngStrtStop_stRefuMod/1 -> A13_AftRun2NetManCal/3(EngStrtStop_stRefuMod)
  VehCfg_stCycCdn/1 -> Subsystem/1(VehCfg_stCycCdn)
  Subsystem/1(HvCoorn_bAuthEna) -> A30_Authcation/Enable
  [GearLvr_stDrvGear] -> A06_ReadyWait2ReadyCal/23(GearLvr_stDrvGear)
  icbcm_stDrvrSeatBelt/1 -> A06_ReadyWait2ReadyCal/24(icbcm_stDrvrSeatBelt)
  icbcm_bStDrvrSeatBeltSigErr/1 -> A06_ReadyWait2ReadyCal/25(icbcm_bStDrvrSeatBeltSigErr)
  icbcm_bDrvrDoorAjar/1 -> A06_ReadyWait2ReadyCal/26(icbcm_bDrvrDoorAjar)
  icbcm_bDrvrDoorAjarSigErr/1 -> A06_ReadyWait2ReadyCal/27(icbcm_bDrvrDoorAjarSigErr)
  A22_ModeBMSReqCal/6(HvCoorn_bRdyLamp) -> HvCoorn_bRdyLamp/1
  A31_VoltModReq/6(HvCoorn_bEngStrt2Dft) -> A32_VoltModSts/6(HvCoorn_bEngStrt2Dft)
  A31_VoltModReq/7(HvCoorn_bHvDisb2Dft) -> A32_VoltModSts/7(HvCoorn_bHvDisb2Dft)
  A31_VoltModReq/8(HvCoorn_bHvDcnct2Dft) -> A32_VoltModSts/8(HvCoorn_bHvDcnct2Dft)
  A31_VoltModReq/9(HvCoorn_bHvReq2Dft) -> A32_VoltModSts/9(HvCoorn_bHvReq2Dft)
  A31_VoltModReq/10(HvCoorn_bVoltModRdy2Dft) -> A32_VoltModSts/10(HvCoorn_bVoltModRdy2Dft)
  A31_VoltModReq/11(HvCoorn_bHvInit2Dft) -> A32_VoltModSts/11(HvCoorn_bHvInit2Dft)
  A31_VoltModReq/12(HvCoorn_bHvCnt2Dft) -> A32_VoltModSts/12(HvCoorn_bHvCnt2Dft)
  A31_VoltModReq/13(HvCoorn_bDCBuck2Dft) -> A32_VoltModSts/13(HvCoorn_bDCBuck2Dft)
  A31_VoltModReq/14(HvCoorn_bHvDcnct2HvInit) -> A32_VoltModSts/14(HvCoorn_bHvDcnct2HvInit)
  A31_VoltModReq/15(HvCoorn_bHvInit2HvCnt) -> A32_VoltModSts/15(HvCoorn_bHvInit2HvCnt)
  A31_VoltModReq/16(HvCoorn_bHvCnt2DCBuck) -> A32_VoltModSts/16(HvCoorn_bHvCnt2DCBuck)
  A31_VoltModReq/17(HvCoorn_bHvInit2EngStrt) -> A32_VoltModSts/17(HvCoorn_bHvInit2EngStrt)
  A31_VoltModReq/18(HvCoorn_bHvCnt2EngStrt) -> A32_VoltModSts/18(HvCoorn_bHvCnt2EngStrt)
  A31_VoltModReq/19(HvCoorn_bDCBuck2EngStrt) -> A32_VoltModSts/19(HvCoorn_bDCBuck2EngStrt)
  [HvCoorn_bStartUpReq] -> A31_VoltModReq/20(HvCoorn_bStartUpReq)
  [HvCoorn_stHVP] -> A31_VoltModReq/21(HvCoorn_stHVP)
  [VehCfg_bFrntMotByp] -> A31_VoltModReq/28(VehCfg_bFrntMotByp)
  [icrm_stMode] -> A31_VoltModReq/26(icrm_stMode)
  [icfm_stMode] -> A31_VoltModReq/25(icfm_stMode)
  [icrm_uAct] -> A31_VoltModReq/30(icrm_uAct)
  [BrkPedDev_bBrk] -> A31_VoltModReq/22(BrkPedDev_bBrk)
  [GearLvr_stDrvGear] -> A31_VoltModReq/23(GearLvr_stDrvGear)
  [VehSpd_vVeh] -> A31_VoltModReq/24(VehSpd_vVeh)
  [icdc_stMode] -> A31_VoltModReq/27(icdc_stMode)
  HvGrid_pwrLoadAct/1 -> A31_VoltModReq/29(HvGrid_pwrLoadAct)
  [HvCoorn_stVoltMod] -> A24_DCDCModeReqCal/4(HvCoorn_stVoltMod)
  HvCoorn_bSocWkupEER/1 -> A01_HighvoltPowerUpReq/96(HvCoorn_bSocWkupEER)
  HvCoorn_bTimerWkupReqEER/1 -> A01_HighvoltPowerUpReq/97(HvCoorn_bTimerWkupReqEER)
  A01_HighvoltPowerUpReq/32(HvCoorn_bSocWkupEEW) -> HvCoorn_bSocWkupEEW/1
  A01_HighvoltPowerUpReq/33(HvCoorn_bTimerWkupReqEEW) -> HvCoorn_bTimerWkupReqEEW/1
  [HvCoorn_stVoltMod] -> A27_ErrCheck/22(HvCoorn_stVoltMod)
  icobc_stV2LFltTyp/1 -> [icobc_stV2LFltTyp], A28_V2L/13(icobc_stV2LFltTyp)
  [icobc_stV2LFltTyp] -> A29_V2In/11(icobc_stV2LFltTyp)
  HvCoorn_stRemLvBatMntnFailRsnEER/1 -> A01_HighvoltPowerUpReq/98(HvCoorn_stRemLvBatMntnFailRsnEER)
  A01_HighvoltPowerUpReq/34(HvCoorn_stRemLvBatMntnFailRsnEEW) -> HvCoorn_stRemLvBatMntnFailRsnEEW/1
  [icicm_bOTAOn] -> A29_V2In/12(icicm_bOTAOn)
  [DTC_bBMSFltLvl6] -> A27_ErrCheck/23(DTC_bBMSFltLvl6)
  DTC_bBMSFltLvlOver5/1 -> Terminator1/1
  icems_bFanAftRunActv/1 -> A01_HighvoltPowerUpReq/99(icems_bFanAftRunActv)
  [ved_bInhbEngStrt] -> A01_HighvoltPowerUpReq/101(ved_bInhbEngStrt)
  RngPrdn_volFuRmnByInstModEEW/1 -> A01_HighvoltPowerUpReq/100(RngPrdn_volFuRmnByInstModEEW)
  idi_bEBSLinWkup/1 -> A01_HighvoltPowerUpReq/102(idi_bEBSLinWkup)
  idi_bTimerWkup/1 -> A01_HighvoltPowerUpReq/103(idi_bTimerWkup)
  HvCoorn_pctHVBatSocEER/1 -> A01_HighvoltPowerUpReq/104(HvCoorn_pctHVBatSocEER)
  idi_noBMSSocCounter/1 -> A01_HighvoltPowerUpReq/105(idi_noBMSSocCounter)
  A01_HighvoltPowerUpReq/35(HvCoorn_pctHVBatSocEEW) -> HvCoorn_pctHVBatSocEEW/1
  A31_VoltModReq/23(HvCoorn_bDft2EngStrtRaw) -> HvCoorn_bDft2EngStrtRaw/1
  [DrvMod_bVehShowMod] -> A01_HighvoltPowerUpReq/106(DrvMod_bVehShowMod)
  A01_HighvoltPowerUpReq/36(HvCoorn_bShowModSocLo) -> HvCoorn_bShowModSocLo/1
  icecc_uPTCAct/1 -> A01_HighvoltPowerUpReq/109(icecc_uPTCAct)
  icecc_uEASAct/1 -> A01_HighvoltPowerUpReq/110(icecc_uEASAct)
  [icisg_uAct] -> A01_HighvoltPowerUpReq/107(icisg_uAct)
  [icrm_uAct] -> A01_HighvoltPowerUpReq/108(icrm_uAct)
  [HvCoorn_bHvRlyOpenAct] -> A02_Init2StupCal/6(HvCoorn_bHvRlyOpenAct)
  ved_bCellVoltUndLimSrus/1 -> A01_HighvoltPowerUpReq/111(ved_bCellVoltUndLimSrus)
